simulink model "IEEE_34_node_2018a"  (R2018a)
settings: Solver=FixedStepDiscrete  StartTime=0.0  StopTime=0.01  RelTol=1e-3
InitFcn:
  | power_34NodeTestFeeder_init;
  | power_34NodeTestFeeder_loads_init;
  | %=============================
  | Vnom_ph_ph = 24900;
  | Vnom = 24900/sqrt(3);
  | Vnom1_ph_ph = 4160;
  | Vnom1 = 4160/sqrt(3);
  | Degrees_ph_ph_gen1 = 0;
  | Frequency = 60;
  | Apparent_power_gen1 = 2500e3;
  | SW1 = 0;
values from neighbouring files (symbols this model uses):
  Pa_802_806 = [1e-6 30 25]*1e3    [power_34NodeTestFeeder_loads_init.m]
  Pa_808_810 = 16e3    (= 16000)    [power_34NodeTestFeeder_loads_init.m]
  Pa_816_824 = [1e-6 5 1e-6]*1e3    [power_34NodeTestFeeder_loads_init.m]
  Pa_818_820 = 34e3    (= 34000)    [power_34NodeTestFeeder_loads_init.m]
  Pa_820_822 = 135e3    (= 135000)    [power_34NodeTestFeeder_loads_init.m]
  Pa_824_826 = 40e3    (= 40000)    [power_34NodeTestFeeder_loads_init.m]
  Pa_824_828 = [1e-6 1e-6 4]*1e3    [power_34NodeTestFeeder_loads_init.m]
  Pa_828_830 = [7 1e-6 1e-6]*1e3    [power_34NodeTestFeeder_loads_init.m]
  Pa_832_858 = [7 2 6]*1e3    [power_34NodeTestFeeder_loads_init.m]
  Pa_834_860 = [16 20 110]*1e3    [power_34NodeTestFeeder_loads_init.m]
  Pa_836_840 = [18 22 1e-6]*1e3    [power_34NodeTestFeeder_loads_init.m]
  Pa_842_844 = [9 1e-6 1e-6]*1e3    [power_34NodeTestFeeder_loads_init.m]
  Pa_844_846 = [1e-6 25 20]*1e3    [power_34NodeTestFeeder_loads_init.m]
  Pa_846_848 = [1e-6 23 1e-6]*1e3    [power_34NodeTestFeeder_loads_init.m]
  Pa_854_856 = 4e3    (= 4000)    [power_34NodeTestFeeder_loads_init.m]
  Pa_858_834 = [4 15 13]*1e3    [power_34NodeTestFeeder_loads_init.m]
  Pa_858_864 = 2e3    (= 2000)    [power_34NodeTestFeeder_loads_init.m]
  Pa_860_836 = [30 10 42]*1e3    [power_34NodeTestFeeder_loads_init.m]
  Pa_862_838 = 28e3    (= 28000)    [power_34NodeTestFeeder_loads_init.m]
  Pp_802_806 = [1e-6 15 14]*1e3    [power_34NodeTestFeeder_loads_init.m]
  Pp_808_810 = 8e3    (= 8000)    [power_34NodeTestFeeder_loads_init.m]
  Pp_816_824 = [1e-6 2 1e-6]*1e3    [power_34NodeTestFeeder_loads_init.m]
  Pp_818_820 = 17e3    (= 17000)    [power_34NodeTestFeeder_loads_init.m]
  Pp_820_822 = 70e3    (= 70000)    [power_34NodeTestFeeder_loads_init.m]
  Pp_824_826 = 20e3    (= 20000)    [power_34NodeTestFeeder_loads_init.m]
  Pp_824_828 = [1e-6 1e-6 2]*1e3    [power_34NodeTestFeeder_loads_init.m]
  Pp_828_830 = [3 1e-6 1e-6]*1e3    [power_34NodeTestFeeder_loads_init.m]
  Pp_832_858 = [3 1 3]*1e3    [power_34NodeTestFeeder_loads_init.m]
  Pp_834_860 = [8 10 55]*1e3    [power_34NodeTestFeeder_loads_init.m]
  Pp_836_840 = [9 11 1e-6]*1e3    [power_34NodeTestFeeder_loads_init.m]
  Pp_842_844 = [5 1e-6 1e-6]*1e3    [power_34NodeTestFeeder_loads_init.m]
  Pp_844_846 = [1e-6 12 11]*1e3    [power_34NodeTestFeeder_loads_init.m]
  Pp_846_848 = [1e-6 11 1e-6]*1e3    [power_34NodeTestFeeder_loads_init.m]
  Pp_854_856 = 2e3    (= 2000)    [power_34NodeTestFeeder_loads_init.m]
  Pp_858_834 = [2 8 7]*1e3    [power_34NodeTestFeeder_loads_init.m]
  Pp_858_864 = 1e3    (= 1000)    [power_34NodeTestFeeder_loads_init.m]
  Pp_860_836 = [15 6 22]*1e3    [power_34NodeTestFeeder_loads_init.m]
  Pp_862_838 = 14e3    (= 14000)    [power_34NodeTestFeeder_loads_init.m]
  V_802_806 = [1.047 1.048 1.048]    [power_34NodeTestFeeder_loads_init.m]
  V_808_810 = 1.014    [power_34NodeTestFeeder_loads_init.m]
  V_816_824 = [1.017 1.025 1.02]*sqrt(3)    [power_34NodeTestFeeder_loads_init.m]
  V_818_820 = 1.016    [power_34NodeTestFeeder_loads_init.m]
  V_820_822 = 0.993    [power_34NodeTestFeeder_loads_init.m]
  V_824_826 = 1.008    [power_34NodeTestFeeder_loads_init.m]
  V_824_828 = [1.008 1.016 1.012]    [power_34NodeTestFeeder_loads_init.m]
  V_828_830 = [1.007 1.015 1.011]    [power_34NodeTestFeeder_loads_init.m]
  V_830 = [0.989 0.998 0.994]*sqrt(3)    [power_34NodeTestFeeder_loads_init.m]
  V_832_858 = [1.036 1.035 1.036]*sqrt(3)    [power_34NodeTestFeeder_loads_init.m]
  V_834_860 = [1.031 1.029 1.031]*sqrt(3)    [power_34NodeTestFeeder_loads_init.m]
  V_836_840 = [1.03 1.029 1.031]*sqrt(3)    [power_34NodeTestFeeder_loads_init.m]
  V_840 = [1.03 1.029 1.031]    [power_34NodeTestFeeder_loads_init.m]
  V_842_844 = [1.031 1.029 1.031]    [power_34NodeTestFeeder_loads_init.m]
  V_844 = [1.031 1.029 1.031]    [power_34NodeTestFeeder_loads_init.m]
  V_844_846 = [1.031 1.029 1.031]    [power_34NodeTestFeeder_loads_init.m]
  V_846_848 = [1.031 1.029 1.031]    [power_34NodeTestFeeder_loads_init.m]
  V_848 = [1.031 1.029 1.031]*sqrt(3)    [power_34NodeTestFeeder_loads_init.m]
  V_854_856 = 0.998    [power_34NodeTestFeeder_loads_init.m]
  V_858_834 = [1.034 1.032 1.034]*sqrt(3)    [power_34NodeTestFeeder_loads_init.m]
  V_860 = [1.03 1.029 1.031]    [power_34NodeTestFeeder_loads_init.m]
  V_860_836 = [1.03 1.029 1.031]*sqrt(3)    [power_34NodeTestFeeder_loads_init.m]
  V_862_838 = 1.029    [power_34NodeTestFeeder_loads_init.m]
  V_890 = [0.917 0.924 0.918]*sqrt(3)    [power_34NodeTestFeeder_loads_init.m]
undefined symbols (not defined in the file or in its folder): Angle, C_300, C_301, C_302, C_303, C_304, Degrees_ph, ft2km, L_300, L_301, L_302, L_303, L_304, Magnitude, ph, ph_gen1, R_300, R_301, R_302, R_303, R_304, Vnom_ph
libraries: powerlib x148
(part 1 of 2)
settings Model: Creator=liyifu  LastModifiedBy=liyifu

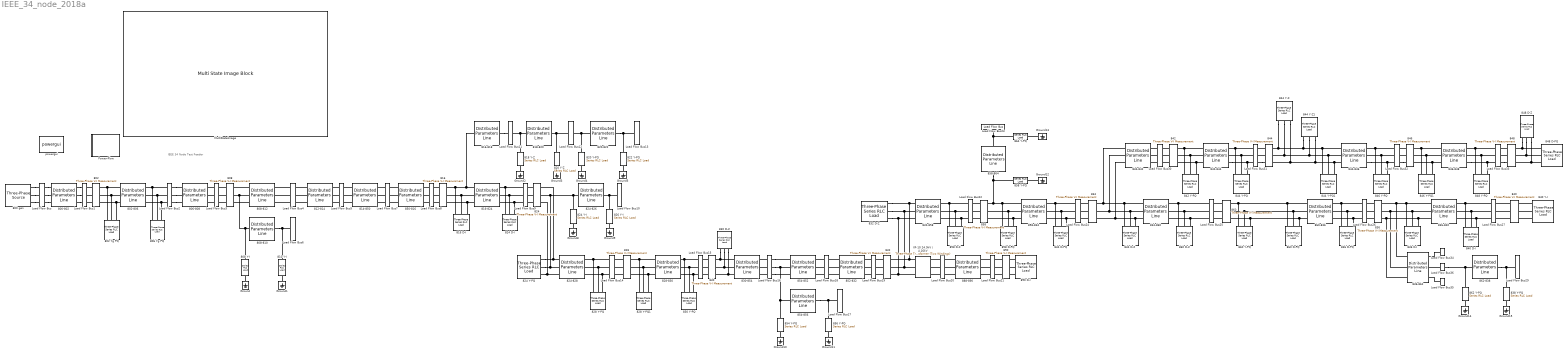
== system IEEE_34_node_2018a ==
  note: IEEE 34 Node Test Feeder
  800 gen : powerlib/Electrical Sources/Three-Phase Source  InternalConnection=Yg  VoltagePhases=on  Voltage=Vnom_ph-ph  PhaseAngle=Degrees_ph-ph_gen1  Voltage_phases=[1.05 1.05 1.05]*Vnom  PhaseAngles_phases=[0 -120 +120]  Frequency=Frequency  NonIdealSource=off  SpecifyImpedance=on  Resistance=0.8929  Inductance=16.58e-3  ShortCircuitLevel=Apparent_power_gen1  BaseVoltage=Vnom_ph_ph  XRratio=8  BusType=swing  Pref=10e3  Qref=0  Prefabc=[10e3, 10e3, 10e3]  Qrefabc=[0, 0, 0]  Qmin=-inf  Qmax=inf
      settings: SourceProductName=Simscape Electrical
  800-802 : powerlib/Elements/Distributed Parameters Line  Phases=3  Frequency=Frequency  Resistance=R_300  Inductance=L_300  Capacitance=C_300  Length=2580*ft2km  x1=[1249.92108084395 26131.4308609001 26009.0181767455;376.991118430775 376.991118430775 376.991118430775;1.94160573810255 0.298080075052811 1.87234868535801]  x2=[1257.44704241073 26098.7880044918 25982.8376072677;376.991118430775 376.991118430775 376.991118430775;1.94920053951311 0.296647201059818 1.87063909565862]  x3=[10.5571233758072 19.865376821896 26.3726391227777;376.991118430775 376.991118430775 376.991118430775;1.91729957078855 -0.988038774966991 0.129228047152116]  x4=[7.52563932812075 151.861194975018 136.408562693795;376.991118430775 376.991118430775 376.991118430775;-1.23536011490698 0.422640409864513 2.06263890147419]  x5=3.46223763231864e-06  V1=ones(3,3)  V2=ones(3,3)  I1=ones(3,3)  I2=ones(3,3)  nHarmo=1  Measurements=None
      settings: SourceProductName=Simscape Electrical
  802 : powerlib/Measurements/Three-Phase V-I Measurement  VoltageMeasurement=phase-to-ground  SetLabelV=on  LabelV=Vabc_802  Vpu=on  VpuLL=off  CurrentMeasurement=yes  SetLabelI=on  LabelI=Iabc_802  Ipu=on  Pbase=100e6  Vbase=Vnom_ph_ph  OutputType=Magnitude-Angle  PhasorSimulation=on  PSBequivalent=0
      settings: SourceProductName=Simscape Electrical
  802 Yg PQ : powerlib/Elements/Three-Phase Series RLC Load  LConnTagsString=A|B|C  Configuration=Y (grounded)  NominalVoltage=[  Vabc=V_802_806*Vnom  Vabcp=[1e3 1e3 1e3]  NominalFrequency=Frequency  UnbalancedPower=on  ActivePower=10e3  InductivePower=100  CapacitivePower=100  Pabc=Pa_802_806/2  QLabc=Pp_802_806/2  QCabc=Pn_802_806  Pabcp=[10e3 9e3 11e3]  QLabcp=[100 90 110]  QCabcp=[100 90 110]  Measurements=None  LoadType=constant PQ
      settings: SourceProductName=Simscape Electrical
      settings: AttributesFormatString=|
      | P= %<Pabc> W
      | Ql=%<QLabc> var
      | Qc=%<QCabc> var
  802-806 : powerlib/Elements/Distributed Parameters Line  Phases=3  Frequency=Frequency  Resistance=R_300  Inductance=L_300  Capacitance=C_300  Length=1730*ft2km  x1=[1257.44704241073 26098.7880044918 25982.8376072677;376.991118430775 376.991118430775 376.991118430775;1.94963055808353 0.297013701686642 1.87099846006617]  x2=[1262.34621488929 26077.2099428151 25966.1115766273;376.991118430775 376.991118430775 376.991118430775;1.95525458709618 0.296060428925334 1.86984860306052]  x3=[11.0972363781312 20.0856417950884 27.4183036232156;376.991118430775 376.991118430775 376.991118430775;1.97949951887063 -0.951655780421584 0.180146149087553]  x4=[8.04996886425621 150.996054293902 135.38429636786;376.991118430775 376.991118430775 376.991118430775;-1.15168297919955 0.422644259105267 2.07252538398702]  x5=2.32157794725242e-06  V1=ones(3,3)  V2=ones(3,3)  I1=ones(3,3)  I2=ones(3,3)  nHarmo=1  Measurements=None
      settings: SourceProductName=Simscape Electrical
  806 Yg PQ : powerlib/Elements/Three-Phase Series RLC Load  LConnTagsString=A|B|C  Configuration=Y (grounded)  NominalVoltage=[  Vabc=V_802_806*Vnom  Vabcp=[1e3 1e3 1e3]  NominalFrequency=Frequency  UnbalancedPower=on  ActivePower=10e3  InductivePower=100  CapacitivePower=100  Pabc=Pa_802_806/2  QLabc=Pp_802_806/2  QCabc=Pn_802_806  Pabcp=[10e3 9e3 11e3]  QLabcp=[100 90 110]  QCabcp=[100 90 110]  Measurements=None  LoadType=constant PQ
      settings: SourceProductName=Simscape Electrical
      settings: AttributesFormatString=|
      | P= %<Pabc> W
      | Ql=%<QLabc> var
      | Qc=%<QCabc> var
  806-808 : powerlib/Elements/Distributed Parameters Line  Phases=3  Frequency=Frequency  Resistance=R_300  Inductance=L_300  Capacitance=C_300  Length=32230*ft2km  x1=[1262.34621488929 26077.2099428151 25966.1115766273;376.991118430775 376.991118430775 376.991118430775;1.93982450898104 0.282909524080493 1.85695376255409]  x2=[1358.17424202311 25682.4173319928 25673.277529669;376.991118430775 376.991118430775 376.991118430775;2.04720135038634 0.265173822183593 1.83534880151853]  x3=[11.6001783263164 20.0026065935591 28.3021789406477;376.991118430775 376.991118430775 376.991118430775;2.01960794152478 -0.945866754158775 0.205483420334985]  x4=[8.46310811689409 146.878902947194 131.899465066813;376.991118430775 376.991118430775 376.991118430775;-1.11000249001825 0.39503335298076 2.05518911486961]  x5=4.32511313525697e-05  V1=ones(3,3)  V2=ones(3,3)  I1=ones(3,3)  I2=ones(3,3)  nHarmo=1  Measurements=None
      settings: SourceProductName=Simscape Electrical
  808 : powerlib/Measurements/Three-Phase V-I Measurement  VoltageMeasurement=phase-to-ground  SetLabelV=on  LabelV=Vabc_808  Vpu=on  VpuLL=off  CurrentMeasurement=yes  SetLabelI=on  LabelI=Iabc_808  Ipu=on  Pbase=100e6  Vbase=Vnom_ph_ph  OutputType=Magnitude-Angle  PhasorSimulation=on  PSBequivalent=0
      settings: SourceProductName=Simscape Electrical
  808 Y-I : powerlib/Elements/Series RLC Load  LConnTagsString=a  RConnTagsString=__new0  NominalVoltage=V_808_810*Vnom  NominalFrequency=Frequency  ActivePower=Pa_808_810/2  InductivePower=Pp_808_810/2  CapacitivePower=Pn_808_810  Setx0=off  InitialVoltage=0  SetiL0=off  InitialCurrent=0  Measurements=None  LoadType=constant I
      settings: SourceProductName=Simscape Electrical
      settings: AttributesFormatString=|
      | P=%<ActivePower> W
      | Ql=%<InductivePower> var
      | Qc=%<CapacitivePower> var
  808-810 : powerlib/Elements/Distributed Parameters Line  Phases=1  Frequency=Frequency  Resistance=R_303(2,2)  Inductance=L_303(2,2)  Capacitance=C_303(2,2)  Length=5804*ft2km  x1=[21119.0815149636;376.991118430775;-2.1231079032275]  x2=[21116.0661432003;376.991118430775;-2.12311859697996]  x3=[34.6870330793776;376.991118430775;-2.11449830893931]  x4=[36.2686607942877;376.991118430775;-2.13404984672294]  x5=7.30496713110932e-06  V1=ones(3,3)  V2=ones(3,3)  I1=ones(3,3)  I2=ones(3,3)  nHarmo=1  Measurements=None
      settings: SourceProductName=Simscape Electrical
  808-812 : powerlib/Elements/Distributed Parameters Line  Phases=3  Frequency=Frequency  Resistance=R_300  Inductance=L_300  Capacitance=C_300  Length=37500*ft2km  x1=[1358.17424202311 25682.4173319928 25673.277529669;376.991118430775 376.991118430775 376.991118430775;2.04453523524972 0.262901518297287 1.83312074219168]  x2=[1469.56545391947 25232.9999723138 25350.7201651836;376.991118430775 376.991118430775 376.991118430775;2.15905513464309 0.24225556988224 1.80744839784332]  x3=[11.6235578223822 19.8498204300557 29.7533327745572;376.991118430775 376.991118430775 376.991118430775;2.12229117690329 -0.959358085491786 0.191726647376344]  x4=[8.24346537921425 143.894679724776 130.199757058103;376.991118430775 376.991118430775 376.991118430775;-1.0079152617316 0.373661075158349 2.04266559454497]  x5=5.03232213999802e-05  V1=ones(3,3)  V2=ones(3,3)  I1=ones(3,3)  I2=ones(3,3)  nHarmo=1  Measurements=None
      settings: SourceProductName=Simscape Electrical
  810 Y-I : powerlib/Elements/Series RLC Load  LConnTagsString=a  RConnTagsString=__new0  NominalVoltage=V_808_810*Vnom  NominalFrequency=Frequency  ActivePower=Pa_808_810/2  InductivePower=Pp_808_810/2  CapacitivePower=Pn_808_810  Setx0=off  InitialVoltage=0  SetiL0=off  InitialCurrent=0  Measurements=None  LoadType=constant I
      settings: SourceProductName=Simscape Electrical
      settings: AttributesFormatString=|
      | P=%<ActivePower> W
      | Ql=%<InductivePower> var
      | Qc=%<CapacitivePower> var
  812-814 : powerlib/Elements/Distributed Parameters Line  Phases=3  Frequency=Frequency  Resistance=R_300  Inductance=L_300  Capacitance=C_300  Length=29730*ft2km  x1=[1469.56545391947 25232.9999723138 25350.7201651836;376.991118430775 376.991118430775 376.991118430775;2.16298601028095 0.245605816788614 1.81073341131004]  x2=[1569.41081620534 24879.7705046649 25102.4809009213;376.991118430775 376.991118430775 376.991118430775;2.24164443153353 0.228987694736397 1.79014174213356]  x3=[11.7818155561854 19.8150927770508 30.4752032611227;376.991118430775 376.991118430775 376.991118430775;2.14520492880805 -1.02022224188866 0.172242125340616]  x4=[8.14305816675558 143.018094733693 129.445364550441;376.991118430775 376.991118430775 376.991118430775;-1.01915035198126 0.362828883761539 2.03152246960354]  x5=3.98962499259043e-05  V1=ones(3,3)  V2=ones(3,3)  I1=ones(3,3)  I2=ones(3,3)  nHarmo=1  Measurements=None
      settings: SourceProductName=Simscape Electrical
  814-850 : powerlib/Elements/Distributed Parameters Line  Phases=3  Frequency=Frequency  Resistance=R_301  Inductance=L_301  Capacitance=C_301  Length=10*ft2km  x1=[669.7608170542 24884.6832259243 25125.0360475112;376.991118430775 376.991118430775 376.991118430775;-1.48243753027906 0.240288742139385 1.79965964476983]  x2=[669.74621388492 24884.491056861 25124.8873333344;376.991118430775 376.991118430775 376.991118430775;-1.4825443216982 0.24028222133131 1.79965138972404]  x3=[10.6357229600782 19.7192063960101 31.0303415847662;376.991118430775 376.991118430775 376.991118430775;2.23998543843376 -1.14786490473853 0.149955273352505]  x4=[11.8856149405288 142.657095608783 128.222738418226;376.991118430775 376.991118430775 376.991118430775;-0.969190911620163 0.376634213985134 2.04330765556362]  x5=1.37899021776565e-08  V1=ones(3,3)  V2=ones(3,3)  I1=ones(3,3)  I2=ones(3,3)  nHarmo=1  Measurements=None
      settings: SourceProductName=Simscape Electrical
  816 : powerlib/Measurements/Three-Phase V-I Measurement  VoltageMeasurement=phase-to-ground  SetLabelV=on  LabelV=Vabc_816  Vpu=on  VpuLL=off  CurrentMeasurement=yes  SetLabelI=on  LabelI=Iabc_816  Ipu=on  Pbase=100e6  Vbase=Vnom_ph_ph  OutputType=Magnitude-Angle  PhasorSimulation=on  PSBequivalent=0
      settings: SourceProductName=Simscape Electrical
  816 D-I : powerlib/Elements/Three-Phase Series RLC Load  LConnTagsString=A|B|C  Configuration=Delta  NominalVoltage=[  Vabc=[1.017 1.025 1.02]*sqrt(3)*Vnom  Vabcp=V_816_824*Vnom  NominalFrequency=Frequency  UnbalancedPower=on  ActivePower=10e3  InductivePower=100  CapacitivePower=100  Pabc=[0 30 25]*1e3/2  QLabc=[0 15 14]*1e3/2  QCabc=[0 0 0]  Pabcp=Pa_816_824/2  QLabcp=Pp_816_824/2  QCabcp=Pn_816_824  Measurements=None  LoadType=constant I
      settings: SourceProductName=Simscape Electrical
      settings: AttributesFormatString=|
      | P= %<Pabc> W
      | Ql=%<QLabc> var
      | Qc=%<QCabc> var
  816-818 : powerlib/Elements/Distributed Parameters Line  Phases=1  Frequency=Frequency  Resistance=R_302(1,1)  Inductance=L_302(1,1)  Capacitance=C_302(1,1)  Length=1710*ft2km  x1=[19869.2600721967;376.991118430775;-0.0627258903807259]  x2=[19851.3152704797;376.991118430775;-0.0627813243909014]  x3=[18.96809714002;376.991118430775;0.328260928650489]  x4=[49.9052646744321;376.991118430775;-0.208674404307824]  x5=2.15222153587128e-06  V1=ones(3,3)  V2=ones(3,3)  I1=ones(3,3)  I2=ones(3,3)  nHarmo=1  Measurements=None
      settings: SourceProductName=Simscape Electrical
  816-824 : powerlib/Elements/Distributed Parameters Line  Phases=3  Frequency=Frequency  Resistance=R_301  Inductance=L_301  Capacitance=C_301  Length=10210*ft2km  x1=[669.297297756189 24878.5341192423 25120.2778264531;376.991118430775 376.991118430775 376.991118430775;-1.49115978603529 0.235758468595441 1.79514164312775]  x2=[637.018239704485 24728.8928242446 24972.8766667643;376.991118430775 376.991118430775 376.991118430775;-1.49783953400905 0.228509227955325 1.7872262979359]  x3=[4.36968691100065 31.1847930023462 28.0632330952332;376.991118430775 376.991118430775 376.991118430775;0.850925211405672 -0.890665928385549 0.228148937955837]  x4=[5.46114690728559 132.850174983932 123.836134516563;376.991118430775 376.991118430775 376.991118430775;-2.10407022380879 0.442934898532415 2.01765281292941]  x5=1.40794901233873e-05  V1=ones(3,3)  V2=ones(3,3)  I1=ones(3,3)  I2=ones(3,3)  nHarmo=1  Measurements=None
      settings: SourceProductName=Simscape Electrical
  818 Y-Z : powerlib/Elements/Series RLC Load  LConnTagsString=a  RConnTagsString=__new0  NominalVoltage=V_818_820*Vnom  NominalFrequency=Frequency  ActivePower=Pa_818_820/2  InductivePower=Pp_818_820/2  CapacitivePower=Pn_818_820  Setx0=off  InitialVoltage=0  SetiL0=off  InitialCurrent=0  Measurements=None  LoadType=constant Z
      settings: SourceProductName=Simscape Electrical
      settings: AttributesFormatString=|
      | P=%<ActivePower> W
      | Ql=%<InductivePower> var
      | Qc=%<CapacitivePower> var
  818-820 : powerlib/Elements/Distributed Parameters Line  Phases=1  Frequency=Frequency  Resistance=R_302(1,1)  Inductance=L_302(1,1)  Capacitance=C_302(1,1)  Length=48150*ft2km  x1=[19851.3152704797;376.991118430775;-0.0848163820973309]  x2=[19391.8214982267;376.991118430775;-0.0858348834112547]  x3=[19.4193208414352;376.991118430775;0.247315554807652]  x4=[46.2735884766118;376.991118430775;-0.238948763434402]  x5=6.06020274574283e-05  V1=ones(3,3)  V2=ones(3,3)  I1=ones(3,3)  I2=ones(3,3)  nHarmo=1  Measurements=None
      settings: SourceProductName=Simscape Electrical
  820 Y-PQ : powerlib/Elements/Series RLC Load  LConnTagsString=a  RConnTagsString=__new0  NominalVoltage=V_820_822*Vnom  NominalFrequency=Frequency  ActivePower=Pa_820_822/2  InductivePower=Pp_820_822/2  CapacitivePower=Pn_820_822  Setx0=off  InitialVoltage=0  SetiL0=off  InitialCurrent=0  Measurements=None  LoadType=constant PQ
      settings: SourceProductName=Simscape Electrical
      settings: AttributesFormatString=|
      | P=%<ActivePower> W
      | Ql=%<InductivePower> var
      | Qc=%<CapacitivePower> var
  820 Y-Z : powerlib/Elements/Series RLC Load  LConnTagsString=a  RConnTagsString=__new0  NominalVoltage=V_818_820*Vnom  NominalFrequency=Frequency  ActivePower=Pa_818_820/2  InductivePower=Pp_818_820/2  CapacitivePower=Pn_818_820  Setx0=off  InitialVoltage=0  SetiL0=off  InitialCurrent=0  Measurements=None  LoadType=constant Z
      settings: SourceProductName=Simscape Electrical
      settings: AttributesFormatString=|
      | P=%<ActivePower> W
      | Ql=%<InductivePower> var
      | Qc=%<CapacitivePower> var
  820-822 : powerlib/Elements/Distributed Parameters Line  Phases=1  Frequency=Frequency  Resistance=R_302(1,1)  Inductance=L_302(1,1)  Capacitance=C_302(1,1)  Length=13740*ft2km  x1=[19391.8214982267;376.991118430775;-0.0695078735990618]  x2=[19332.7468483932;376.991118430775;-0.0695769850406438]  x3=[26.2226131335753;376.991118430775;0.048560985296662]  x4=[38.8103545088805;376.991118430775;-0.154709382906807]  x5=1.72932888320886e-05  V1=ones(3,3)  V2=ones(3,3)  I1=ones(3,3)  I2=ones(3,3)  nHarmo=1  Measurements=None
      settings: SourceProductName=Simscape Electrical
  822 Y-PQ : powerlib/Elements/Series RLC Load  LConnTagsString=a  RConnTagsString=__new0  NominalVoltage=V_820_822*Vnom  NominalFrequency=Frequency  ActivePower=Pa_820_822/2  InductivePower=Pp_820_822/2  CapacitivePower=Pn_820_822  Setx0=off  InitialVoltage=0  SetiL0=off  InitialCurrent=0  Measurements=None  LoadType=constant PQ
      settings: SourceProductName=Simscape Electrical
      settings: AttributesFormatString=|
      | P=%<ActivePower> W
      | Ql=%<InductivePower> var
      | Qc=%<CapacitivePower> var
  824 : powerlib/Measurements/Three-Phase V-I Measurement  VoltageMeasurement=phase-to-ground  SetLabelV=on  LabelV=Vabc_824  Vpu=on  VpuLL=off  CurrentMeasurement=yes  SetLabelI=on  LabelI=Iabc_824  Ipu=on  Pbase=100e6  Vbase=Vnom_ph_ph  OutputType=Magnitude-Angle  PhasorSimulation=on  PSBequivalent=0
      settings: SourceProductName=Simscape Electrical
  824 D-I : powerlib/Elements/Three-Phase Series RLC Load  LConnTagsString=A|B|C  Configuration=Delta  NominalVoltage=[  Vabc=[1.017 1.025 1.02]*sqrt(3)*Vnom  Vabcp=V_816_824*Vnom  NominalFrequency=Frequency  UnbalancedPower=on  ActivePower=10e3  InductivePower=100  CapacitivePower=100  Pabc=[0 30 25]*1e3/2  QLabc=[0 15 14]*1e3/2  QCabc=[0 0 0]  Pabcp=Pa_816_824/2  QLabcp=Pp_816_824/2  QCabcp=Pn_816_824  Measurements=None  LoadType=constant I
      settings: SourceProductName=Simscape Electrical
      settings: AttributesFormatString=|
      | P= %<Pabc> W
      | Ql=%<QLabc> var
      | Qc=%<QCabc> var
  824 Y-I : powerlib/Elements/Series RLC Load  LConnTagsString=a  RConnTagsString=__new0  NominalVoltage=V_824_826*Vnom  NominalFrequency=Frequency  ActivePower=Pa_824_826/2  InductivePower=Pp_824_826/2  CapacitivePower=Pn_824_826  Setx0=off  InitialVoltage=0  SetiL0=off  InitialCurrent=0  Measurements=None  LoadType=constant I
      settings: SourceProductName=Simscape Electrical
      settings: AttributesFormatString=|
      | P=%<ActivePower> W
      | Ql=%<InductivePower> var
      | Qc=%<CapacitivePower> var
  824 Y-PQ : powerlib/Elements/Three-Phase Series RLC Load  LConnTagsString=A|B|C  Configuration=Y (grounded)  NominalVoltage=[  Vabc=V_824_828*Vnom  Vabcp=[1.008 1.016 1.012]*Vnom  NominalFrequency=Frequency  UnbalancedPower=on  ActivePower=10e3  InductivePower=100  CapacitivePower=100  Pabc=Pa_824_828/2  QLabc=Pp_824_828/2  QCabc=Pn_824_828  Pabcp=[0 0 4]*1e3/2  QLabcp=[0 0 2]*1e3/2  QCabcp=[0 0 0]  Measurements=None  LoadType=constant PQ
      settings: SourceProductName=Simscape Electrical
      settings: AttributesFormatString=|
      | P= %<Pabc> W
      | Ql=%<QLabc> var
      | Qc=%<QCabc> var
  824-826 : powerlib/Elements/Distributed Parameters Line  Phases=1  Frequency=Frequency  Resistance=R_303(2,2)  Inductance=L_303(2,2)  Capacitance=C_303(2,2)  Length=3030*ft2km  x1=[20638.2047774201;376.991118430775;-2.17740572018252]  x2=[20634.23117712;376.991118430775;-2.1774123534692]  x3=[32.7859887350078;376.991118430775;-2.14899511081035]  x4=[36.7043804950352;376.991118430775;-2.20415074648027]  x5=3.81358552847368e-06  V1=ones(3,3)  V2=ones(3,3)  I1=ones(3,3)  I2=ones(3,3)  nHarmo=1  Measurements=None
      settings: SourceProductName=Simscape Electrical
  824-828 : powerlib/Elements/Distributed Parameters Line  Phases=3  Frequency=Frequency  Resistance=R_301  Inductance=L_301  Capacitance=C_301  Length=840*ft2km  x1=[637.018239704485 24728.8928242446 24972.8766667643;376.991118430775 376.991118430775 376.991118430775;-1.49296837961468 0.2324791474979 1.79113396244307]  x2=[635.673675429622 24717.2262249166 24961.4172077253;376.991118430775 376.991118430775 376.991118430775;-1.49430047635018 0.23190162251329 1.79046003567284]  x3=[2.25223495446006 31.9396656829298 30.8215706689758;376.991118430775 376.991118430775 376.991118430775;1.30619849621643 -0.81398677567269 0.255650052760832]  x4=[3.59155607107433 130.840713390775 123.949302221309;376.991118430775 376.991118430775 376.991118430775;-1.70546632028145 0.444876316743132 2.04175653602867]  x5=1.15835178292315e-06  V1=ones(3,3)  V2=ones(3,3)  I1=ones(3,3)  I2=ones(3,3)  nHarmo=1  Measurements=None
      settings: SourceProductName=Simscape Electrical
  826 Y-I : powerlib/Elements/Series RLC Load  LConnTagsString=a  RConnTagsString=__new0  NominalVoltage=V_824_826*Vnom  NominalFrequency=Frequency  ActivePower=Pa_824_826/2  InductivePower=Pp_824_826/2  CapacitivePower=Pn_824_826  Setx0=off  InitialVoltage=0  SetiL0=off  InitialCurrent=0  Measurements=None  LoadType=constant I
      settings: SourceProductName=Simscape Electrical
      settings: AttributesFormatString=|
      | P=%<ActivePower> W
      | Ql=%<InductivePower> var
      | Qc=%<CapacitivePower> var
  828 : powerlib/Measurements/Three-Phase V-I Measurement  VoltageMeasurement=phase-to-ground  SetLabelV=on  LabelV=Vabc_828  Vpu=on  VpuLL=off  CurrentMeasurement=yes  SetLabelI=on  LabelI=Iabc_828  Ipu=on  Pbase=100e6  Vbase=Vnom_ph_ph  OutputType=Magnitude-Angle  PhasorSimulation=on  PSBequivalent=0
      settings: SourceProductName=Simscape Electrical
  828 Y-PQ : powerlib/Elements/Three-Phase Series RLC Load  LConnTagsString=A|B|C  Configuration=Y (grounded)  NominalVoltage=[  Vabc=V_824_828*Vnom  Vabcp=[1.008 1.016 1.012]*Vnom  NominalFrequency=Frequency  UnbalancedPower=on  ActivePower=10e3  InductivePower=100  CapacitivePower=100  Pabc=Pa_824_828/2  QLabc=Pp_824_828/2  QCabc=Pn_824_828  Pabcp=[0 0 4]*1e3/2  QLabcp=[0 0 2]*1e3/2  QCabcp=[0 0 0]  Measurements=None  LoadType=constant PQ
      settings: SourceProductName=Simscape Electrical
      settings: AttributesFormatString=|
      | P= %<Pabc> W
      | Ql=%<QLabc> var
      | Qc=%<QCabc> var
  828 Y-PQ1 : powerlib/Elements/Three-Phase Series RLC Load  LConnTagsString=A|B|C  Configuration=Y (grounded)  NominalVoltage=[  Vabc=V_828_830*Vnom  Vabcp=[1.008 1.016 1.012]*Vnom  NominalFrequency=Frequency  UnbalancedPower=on  ActivePower=10e3  InductivePower=100  CapacitivePower=100  Pabc=Pa_828_830/2  QLabc=Pp_828_830/2  QCabc=Pn_828_830  Pabcp=[0 0 4]*1e3/2  QLabcp=[0 0 2]*1e3/2  QCabcp=[0 0 0]  Measurements=None  LoadType=constant PQ
      settings: SourceProductName=Simscape Electrical
      settings: AttributesFormatString=|
      | P= %<Pabc> W
      | Ql=%<QLabc> var
      | Qc=%<QCabc> var
  828-830 : powerlib/Elements/Distributed Parameters Line  Phases=3  Frequency=Frequency  Resistance=R_301  Inductance=L_301  Capacitance=C_301  Length=20440*ft2km  x1=[635.673675429622 24717.2262249166 24961.4172077253;376.991118430775 376.991118430775 376.991118430775;-1.50448987081439 0.223597415145683 1.78228605228538]  x2=[601.287036352134 24436.8994336664 24686.5156314332;376.991118430775 376.991118430775 376.991118430775;-1.53587251532522 0.209428113553337 1.76580414802682]  x3=[2.31969871934651 31.7720570459509 30.5873085234824;376.991118430775 376.991118430775 376.991118430775;1.21736133349944 -0.830325240506862 0.24642590112485]  x4=[3.59292222973066 128.054918862299 121.560613327383;376.991118430775 376.991118430775 376.991118430775;-1.77870237402968 0.428167673220865 2.02387530834998]  x5=2.81865600511299e-05  V1=ones(3,3)  V2=ones(3,3)  I1=ones(3,3)  I2=ones(3,3)  nHarmo=1  Measurements=None
      settings: SourceProductName=Simscape Electrical
  830 : powerlib/Measurements/Three-Phase V-I Measurement  VoltageMeasurement=phase-to-ground  SetLabelV=on  LabelV=Vabc_830  Vpu=on  VpuLL=off  CurrentMeasurement=yes  SetLabelI=on  LabelI=Iabc_830  Ipu=on  Pbase=100e6  Vbase=Vnom_ph_ph  OutputType=Magnitude-Angle  PhasorSimulation=on  PSBequivalent=0
      settings: SourceProductName=Simscape Electrical
  830 D-Z : powerlib/Elements/Three-Phase Series RLC Load  LConnTagsString=A|B|C  Configuration=Delta  NominalVoltage=[  Vabc=[1.017 1.025 1.02]*sqrt(3)*Vnom  Vabcp=V_830*Vnom  NominalFrequency=Frequency  UnbalancedPower=on  ActivePower=10e3  InductivePower=100  CapacitivePower=100  Pabc=[0 30 25]*1e3/2  QLabc=[0 15 14]*1e3/2  QCabc=[0 0 0]  Pabcp=Pa_830  QLabcp=Pp_830  QCabcp=Pn_830  Measurements=None  LoadType=constant Z
      settings: SourceProductName=Simscape Electrical
      settings: AttributesFormatString=|
      | P= %<Pabc> W
      | Ql=%<QLabc> var
      | Qc=%<QCabc> var
  830 Y-PQ : powerlib/Elements/Three-Phase Series RLC Load  LConnTagsString=A|B|C  Configuration=Y (grounded)  NominalVoltage=[  Vabc=V_828_830*Vnom  Vabcp=[1.008 1.016 1.012]*Vnom  NominalFrequency=Frequency  UnbalancedPower=on  ActivePower=10e3  InductivePower=100  CapacitivePower=100  Pabc=Pa_828_830/2  QLabc=Pp_828_830/2  QCabc=Pn_828_830  Pabcp=[0 0 4]*1e3/2  QLabcp=[0 0 2]*1e3/2  QCabcp=[0 0 0]  Measurements=None  LoadType=constant PQ
      settings: SourceProductName=Simscape Electrical
      settings: AttributesFormatString=|
      | P= %<Pabc> W
      | Ql=%<QLabc> var
      | Qc=%<QCabc> var
  830-854 : powerlib/Elements/Distributed Parameters Line  Phases=3  Frequency=Frequency  Resistance=R_301  Inductance=L_301  Capacitance=C_301  Length=520*ft2km  x1=[601.287036352134 24436.8994336664 24686.5156314332;376.991118430775 376.991118430775 376.991118430775;-1.52551676340037 0.217867899816742 1.77411158420428]  x2=[600.415344439585 24430.2182967214 24679.9493391831;376.991118430775 376.991118430775 376.991118430775;-1.52617739951622 0.217500171996073 1.77369575342487]  x3=[2.24837479458079 34.3986849322115 31.5997630877242;376.991118430775 376.991118430775 376.991118430775;1.10573653139527 -0.8187450702249 0.306471269019442]  x4=[3.4533394454739 128.179899166488 120.709427985989;376.991118430775 376.991118430775 376.991118430775;-1.84935582786226 0.450612810902678 2.03721471359926]  x5=7.17074913238139e-07  V1=ones(3,3)  V2=ones(3,3)  I1=ones(3,3)  I2=ones(3,3)  nHarmo=1  Measurements=None
      settings: SourceProductName=Simscape Electrical
  832 : powerlib/Measurements/Three-Phase V-I Measurement  VoltageMeasurement=phase-to-ground  SetLabelV=on  LabelV=Vabc_832  Vpu=on  VpuLL=off  CurrentMeasurement=yes  SetLabelI=on  LabelI=Iabc_832  Ipu=on  Pbase=100e6  Vbase=Vnom_ph_ph  OutputType=Magnitude-Angle  PhasorSimulation=on  PSBequivalent=0
      settings: SourceProductName=Simscape Electrical
  832 D-Z : powerlib/Elements/Three-Phase Series RLC Load  LConnTagsString=A|B|C  Configuration=Delta  NominalVoltage=[  Vabc=[1.017 1.025 1.02]*sqrt(3)*Vnom  Vabcp=V_832_858*Vnom  NominalFrequency=Frequency  UnbalancedPower=on  ActivePower=10e3  InductivePower=100  CapacitivePower=100  Pabc=[0 30 25]*1e3/2  QLabc=[0 15 14]*1e3/2  QCabc=[0 0 0]  Pabcp=Pa_832_858/2  QLabcp=Pp_832_858/2  QCabcp=Pn_832_858  Measurements=None  LoadType=constant Z
      settings: SourceProductName=Simscape Electrical
      settings: AttributesFormatString=|
      | P= %<Pabc> W
      | Ql=%<QLabc> var
      | Qc=%<QCabc> var
  832-858 : powerlib/Elements/Distributed Parameters Line  Phases=3  Frequency=Frequency  Resistance=R_301  Inductance=L_301  Capacitance=C_301  Length=4900*ft2km  x1=[544.297090319122 23962.1950623007 24225.8849285826;376.991118430775 376.991118430775 376.991118430775;-1.57363040145649 0.189493419417186 1.74208300295025]  x2=[538.916079582122 23936.381353331 24203.4007325891;376.991118430775 376.991118430775 376.991118430775;-1.57527517916447 0.185868800435926 1.73805296350572]  x3=[1.29723917616971 52.8684457924366 47.3954754221382;376.991118430775 376.991118430775 376.991118430775;0.622930723400035 -0.656927709691266 0.637340252599691]  x4=[2.20825884422358 111.101810545025 104.723116464672;376.991118430775 376.991118430775 376.991118430775;-2.07115911053738 0.550064652386419 2.15459413769142]  x5=6.7570520670517e-06  V1=ones(3,3)  V2=ones(3,3)  I1=ones(3,3)  I2=ones(3,3)  nHarmo=1  Measurements=None
      settings: SourceProductName=Simscape Electrical
  834 : powerlib/Measurements/Three-Phase V-I Measurement  VoltageMeasurement=phase-to-ground  SetLabelV=on  LabelV=Vabc_834  Vpu=on  VpuLL=off  CurrentMeasurement=yes  SetLabelI=on  LabelI=Iabc_834  Ipu=on  Pbase=100e6  Vbase=Vnom_ph_ph  OutputType=Magnitude-Angle  PhasorSimulation=on  PSBequivalent=0
      settings: SourceProductName=Simscape Electrical
  834 D-PQ : powerlib/Elements/Three-Phase Series RLC Load  LConnTagsString=A|B|C  Configuration=Delta  NominalVoltage=[  Vabc=[1.017 1.025 1.02]*sqrt(3)*Vnom  Vabcp=V_858_834*Vnom  NominalFrequency=Frequency  UnbalancedPower=on  ActivePower=10e3  InductivePower=100  CapacitivePower=100  Pabc=[0 30 25]*1e3/2  QLabc=[0 15 14]*1e3/2  QCabc=[0 0 0]  Pabcp=Pa_858_834/2  QLabcp=Pp_858_834/2  QCabcp=Pn_858_834  Measurements=None  LoadType=constant PQ
      settings: SourceProductName=Simscape Electrical
      settings: AttributesFormatString=|
      | P= %<Pabc> W
      | Ql=%<QLabc> var
      | Qc=%<QCabc> var
  834 D-Z : powerlib/Elements/Three-Phase Series RLC Load  LConnTagsString=A|B|C  Configuration=Delta  NominalVoltage=[  Vabc=[1.017 1.025 1.02]*sqrt(3)*Vnom  Vabcp=V_834_860*Vnom  NominalFrequency=Frequency  UnbalancedPower=on  ActivePower=10e3  InductivePower=100  CapacitivePower=100  Pabc=[0 30 25]*1e3/2  QLabc=[0 15 14]*1e3/2  QCabc=[0 0 0]  Pabcp=Pa_834_860/2  QLabcp=Pp_834_860/2  QCabcp=Pn_834_860  Measurements=None  LoadType=constant Z
      settings: SourceProductName=Simscape Electrical
      settings: AttributesFormatString=|
      | P= %<Pabc> W
      | Ql=%<QLabc> var
      | Qc=%<QCabc> var
  834-842 : powerlib/Elements/Distributed Parameters Line  Phases=3  Frequency=Frequency  Resistance=R_301  Inductance=L_301  Capacitance=C_301  Length=280*ft2km  x1=[532.488097890621 23907.9048332495 24179.347575776;376.991118430775 376.991118430775 376.991118430775;-1.5738010972037 0.183503521668224 1.73519817574279]  x2=[532.560098856686 23908.1567468527 24179.8968067617;376.991118430775 376.991118430775 376.991118430775;-1.57375382845556 0.183279337224048 1.73497886153928]  x3=[0.972485409830439 70.724344430212 62.0978591081052;376.991118430775 376.991118430775 376.991118430775;-1.77765362434399 -0.614329731124174 0.834703061723499]  x4=[0.288188518469659 103.091898225527 92.6081132341689;376.991118430775 376.991118430775 376.991118430775;-0.822017371184678 0.696581277115551 2.28820569141929]  x5=3.86117260974383e-07  V1=ones(3,3)  V2=ones(3,3)  I1=ones(3,3)  I2=ones(3,3)  nHarmo=1  Measurements=None
      settings: SourceProductName=Simscape Electrical
  834-860 : powerlib/Elements/Distributed Parameters Line  Phases=3  Frequency=Frequency  Resistance=R_301  Inductance=L_301  Capacitance=C_301  Length=2020*ft2km  x1=[532.488097890621 23907.9048332495 24179.347575776;376.991118430775 376.991118430775 376.991118430775;-1.57470566589593 0.182766311422324 1.73447252619717]  x2=[529.898068973042 23898.4588495649 24170.0388321035;376.991118430775 376.991118430775 376.991118430775;-1.57474565502375 0.182826368932349 1.73445969410462]  x3=[1.63328036165873 58.7099677379436 47.5606280616576;376.991118430775 376.991118430775 376.991118430775;0.488910014175005 0.307610071221618 1.85359151611361]  x4=[2.40930708204933 81.0863982856748 70.2473653685472;376.991118430775 376.991118430775 376.991118430775;-2.21508285043218 0.0918009452492619 1.65321083575864]  x5=2.78556023988662e-06  V1=ones(3,3)  V2=ones(3,3)  I1=ones(3,3)  I2=ones(3,3)  nHarmo=1  Measurements=None
      settings: SourceProductName=Simscape Electrical
  836 : powerlib/Measurements/Three-Phase V-I Measurement  VoltageMeasurement=phase-to-ground  SetLabelV=on  LabelV=Vabc_836  Vpu=on  VpuLL=off  CurrentMeasurement=yes  SetLabelI=on  LabelI=Iabc_836  Ipu=on  Pbase=100e6  Vbase=Vnom_ph_ph  OutputType=Magnitude-Angle  PhasorSimulation=on  PSBequivalent=0
      settings: SourceProductName=Simscape Electrical
  836 D-I : powerlib/Elements/Three-Phase Series RLC Load  LConnTagsString=A|B|C  Configuration=Delta  NominalVoltage=[  Vabc=[1.017 1.025 1.02]*sqrt(3)*Vnom  Vabcp=V_836_840*Vnom  NominalFrequency=Frequency  UnbalancedPower=on  ActivePower=10e3  InductivePower=100  CapacitivePower=100  Pabc=[0 30 25]*1e3/2  QLabc=[0 15 14]*1e3/2  QCabc=[0 0 0]  Pabcp=Pa_836_840/2  QLabcp=Pp_836_840/2  QCabcp=Pn_836_840  Measurements=None  LoadType=constant I
      settings: SourceProductName=Simscape Electrical
      settings: AttributesFormatString=|
      | P= %<Pabc> W
      | Ql=%<QLabc> var
      | Qc=%<QCabc> var
  836 D-PQ : powerlib/Elements/Three-Phase Series RLC Load  LConnTagsString=A|B|C  Configuration=Delta  NominalVoltage=[  Vabc=[1.017 1.025 1.02]*sqrt(3)*Vnom  Vabcp=V_860_836*Vnom  NominalFrequency=Frequency  UnbalancedPower=on  ActivePower=10e3  InductivePower=100  CapacitivePower=100  Pabc=[0 30 25]*1e3/2  QLabc=[0 15 14]*1e3/2  QCabc=[0 0 0]  Pabcp=Pa_860_836/2  QLabcp=Pp_860_836/2  QCabcp=Pn_860_836  Measurements=None  LoadType=constant PQ
      settings: SourceProductName=Simscape Electrical
      settings: AttributesFormatString=|
      | P= %<Pabc> W
      | Ql=%<QLabc> var
      | Qc=%<QCabc> var
  836-840 : powerlib/Elements/Distributed Parameters Line  Phases=3  Frequency=Frequency  Resistance=R_301  Inductance=L_301  Capacitance=C_301  Length=860*ft2km  x1=[526.843358587077 23892.7809998017 24164.7359964069;376.991118430775 376.991118430775 376.991118430775;-1.57308914165041 0.183273286351239 1.73500447386127]  x2=[526.803514703196 23892.1759032398 24164.0726411531;376.991118430775 376.991118430775 376.991118430775;-1.57311376940977 0.183271808368671 1.73501207127654]  x3=[0.510845372924359 67.6621593415957 57.059033430526;376.991118430775 376.991118430775 376.991118430775;-1.5015887629287 0.193756770923144 1.76168035684478]  x4=[0.64168752557632 71.3999314397603 60.2490456702427;376.991118430775 376.991118430775 376.991118430775;-1.63041606492187 0.172982288304378 1.70939949530344]  x5=1.18593158727846e-06  V1=ones(3,3)  V2=ones(3,3)  I1=ones(3,3)  I2=ones(3,3)  nHarmo=1  Measurements=None
      settings: SourceProductName=Simscape Electrical
  836-862 : powerlib/Elements/Distributed Parameters Line  Phases=3  Frequency=Frequency  Resistance=R_301  Inductance=L_301  Capacitance=C_301  Length=280*ft2km  x1=[526.843358587077 23892.7809998017 24164.7359964069;376.991118430775 376.991118430775 376.991118430775;-1.572787618753 0.183519023099872 1.73524635704314]  x2=[526.548353531827 23892.6530875428 24164.6254067925;376.991118430775 376.991118430775 376.991118430775;-1.57263196771958 0.183514334830567 1.73525075784239]  x3=[1.5114465772424 67.9042329654386 58.2102323915336;376.991118430775 376.991118430775 376.991118430775;0.128516773467724 0.176124880592363 1.75998009197564]  x4=[2.01487486252301 71.211679623214 59.1340381995524;376.991118430775 376.991118430775 376.991118430775;-2.41146845447374 0.190449273339831 1.71078759688826]  x5=3.86117260974383e-07  V1=ones(3,3)  V2=ones(3,3)  I1=ones(3,3)  I2=ones(3,3)  nHarmo=1  Measurements=None
      settings: SourceProductName=Simscape Electrical
  838 Y-PQ : powerlib/Elements/Series RLC Load  LConnTagsString=a  RConnTagsString=__new0  NominalVoltage=V_862_838*Vnom  NominalFrequency=Frequency  ActivePower=Pa_862_838/2  InductivePower=Pp_862_838/2  CapacitivePower=Pn_862_838  Setx0=off  InitialVoltage=0  SetiL0=off  InitialCurrent=0  Measurements=None  LoadType=constant PQ
      settings: SourceProductName=Simscape Electrical
      settings: AttributesFormatString=|
      | P=%<ActivePower> W
      | Ql=%<InductivePower> var
      | Qc=%<CapacitivePower> var
  840 : powerlib/Measurements/Three-Phase V-I Measurement  VoltageMeasurement=phase-to-ground  SetLabelV=on  LabelV=Vabc_840  Vpu=on  VpuLL=off  CurrentMeasurement=yes  SetLabelI=on  LabelI=Iabc_840  Ipu=on  Pbase=100e6  Vbase=Vnom_ph_ph  OutputType=Magnitude-Angle  PhasorSimulation=on  PSBequivalent=0
      settings: SourceProductName=Simscape Electrical
  840 D-I : powerlib/Elements/Three-Phase Series RLC Load  LConnTagsString=A|B|C  Configuration=Delta  NominalVoltage=[  Vabc=[1.017 1.025 1.02]*sqrt(3)*Vnom  Vabcp=V_836_840*Vnom  NominalFrequency=Frequency  UnbalancedPower=on  ActivePower=10e3  InductivePower=100  CapacitivePower=100  Pabc=[0 30 25]*1e3/2  QLabc=[0 15 14]*1e3/2  QCabc=[0 0 0]  Pabcp=Pa_836_840/2  QLabcp=Pp_836_840/2  QCabcp=Pn_836_840  Measurements=None  LoadType=constant I
      settings: SourceProductName=Simscape Electrical
      settings: AttributesFormatString=|
      | P= %<Pabc> W
      | Ql=%<QLabc> var
      | Qc=%<QCabc> var
  840 Y-I : powerlib/Elements/Three-Phase Series RLC Load  LConnTagsString=A|B|C  Configuration=Y (grounded)  NominalVoltage=1000  Vabc=V_840*Vnom  Vabcp=[1e3 1e3 1e3]  NominalFrequency=Frequency  UnbalancedPower=on  ActivePower=10e3  InductivePower=100  CapacitivePower=100  Pabc=Pa_840  QLabc=Pp_840  QCabc=Pn_840  Pabcp=[10e3 9e3 11e3]  QLabcp=[100 90 110]  QCabcp=[100 90 110]  Measurements=None  LoadType=constant I
      settings: SourceProductName=Simscape Electrical
      settings: AttributesFormatString=|
      | P= %<Pabc> W
      | Ql=%<QLabc> var
      | Qc=%<QCabc> var
  842 : powerlib/Measurements/Three-Phase V-I Measurement  VoltageMeasurement=phase-to-ground  SetLabelV=on  LabelV=Vabc_842  Vpu=on  VpuLL=off  CurrentMeasurement=yes  SetLabelI=on  LabelI=Iabc_842  Ipu=on  Pbase=100e6  Vbase=Vnom_ph_ph  OutputType=Magnitude-Angle  PhasorSimulation=on  PSBequivalent=0
      settings: SourceProductName=Simscape Electrical
  842 Y-PQ : powerlib/Elements/Three-Phase Series RLC Load  LConnTagsString=A|B|C  Configuration=Y (grounded)  NominalVoltage=[  Vabc=V_842_844*Vnom  Vabcp=[1.031 1.029 1.031]*sqrt(3)*Vnom  NominalFrequency=Frequency  UnbalancedPower=on  ActivePower=10e3  InductivePower=100  CapacitivePower=100  Pabc=Pa_842_844/2  QLabc=Pp_842_844/2  QCabc=Pn_842_844  Pabcp=[16 20 110]*1e3/2  QLabcp=[8 10 55]*1e3/2  QCabcp=[0 0 0]  Measurements=None  LoadType=constant PQ
      settings: SourceProductName=Simscape Electrical
      settings: AttributesFormatString=|
      | P= %<Pabc> W
      | Ql=%<QLabc> var
      | Qc=%<QCabc> var
  842-844 : powerlib/Elements/Distributed Parameters Line  Phases=3  Frequency=Frequency  Resistance=R_301  Inductance=L_301  Capacitance=C_301  Length=1350*ft2km  x1=[532.560098856686 23908.1567468527 24179.8968067617;376.991118430775 376.991118430775 376.991118430775;-1.57431008621457 0.182825995291225 1.73453262877272]  x2=[532.858804830353 23909.5344403469 24182.5702844361;376.991118430775 376.991118430775 376.991118430775;-1.57364231122933 0.18174309367146 1.73347760584717]  x3=[1.11121270955152 71.024975502821 62.0592829213778;376.991118430775 376.991118430775 376.991118430775;-1.55136832727018 -0.61506623607051 0.835624985905007]  x4=[0.0578291861142763 102.887673684504 92.4200514058512;376.991118430775 376.991118430775 376.991118430775;-2.03117715282753 0.698439307112783 2.28667687424365]  x5=1.86163679398363e-06  V1=ones(3,3)  V2=ones(3,3)  I1=ones(3,3)  I2=ones(3,3)  nHarmo=1  Measurements=None
      settings: SourceProductName=Simscape Electrical
  844 : powerlib/Measurements/Three-Phase V-I Measurement  VoltageMeasurement=phase-to-ground  SetLabelV=on  LabelV=Vabc_844  Vpu=on  VpuLL=off  CurrentMeasurement=yes  SetLabelI=on  LabelI=Iabc_844  Ipu=on  Pbase=100e6  Vbase=Vnom_ph_ph  OutputType=Magnitude-Angle  PhasorSimulation=on  PSBequivalent=0
      settings: SourceProductName=Simscape Electrical
  844 Y-PQ : powerlib/Elements/Three-Phase Series RLC Load  LConnTagsString=A|B|C  Configuration=Y (grounded)  NominalVoltage=[  Vabc=V_842_844*Vnom  Vabcp=[1.031 1.029 1.031]*sqrt(3)*Vnom  NominalFrequency=Frequency  UnbalancedPower=on  ActivePower=10e3  InductivePower=100  CapacitivePower=100  Pabc=Pa_842_844/2  QLabc=Pp_842_844/2  QCabc=Pn_842_844  Pabcp=[16 20 110]*1e3/2  QLabcp=[8 10 55]*1e3/2  QCabcp=[0 0 0]  Measurements=None  LoadType=constant PQ
      settings: SourceProductName=Simscape Electrical
      settings: AttributesFormatString=|
      | P= %<Pabc> W
      | Ql=%<QLabc> var
      | Qc=%<QCabc> var
  844 Y-PQ1 : powerlib/Elements/Three-Phase Series RLC Load  LConnTagsString=A|B|C  Configuration=Y (grounded)  NominalVoltage=[  Vabc=V_844_846*Vnom  Vabcp=[1.031 1.029 1.031]*sqrt(3)*Vnom  NominalFrequency=Frequency  UnbalancedPower=on  ActivePower=10e3  InductivePower=100  CapacitivePower=100  Pabc=Pa_844_846/2  QLabc=Pp_844_846/2  QCabc=Pn_844_846  Pabcp=[16 20 110]*1e3/2  QLabcp=[8 10 55]*1e3/2  QCabcp=[0 0 0]  Measurements=None  LoadType=constant PQ
      settings: SourceProductName=Simscape Electrical
      settings: AttributesFormatString=|
      | P= %<Pabc> W
      | Ql=%<QLabc> var
      | Qc=%<QCabc> var
  844 Y-Z : powerlib/Elements/Three-Phase Series RLC Load  LConnTagsString=A|B|C  Configuration=Y (grounded)  NominalVoltage=[  Vabc=V_844*Vnom  Vabcp=[1.031 1.029 1.031]*sqrt(3)*Vnom  NominalFrequency=Frequency  UnbalancedPower=on  ActivePower=10e3  InductivePower=100  CapacitivePower=100  Pabc=Pa_844  QLabc=Pp_844  QCabc=[0 0 0]  Pabcp=[16 20 110]*1e3/2  QLabcp=[8 10 55]*1e3/2  QCabcp=[0 0 0]  Measurements=Branch voltages and currents  LoadType=constant Z
      settings: SourceProductName=Simscape Electrical
      settings: AttributesFormatString=|
      | P= %<Pabc> W
      | Ql=%<QLabc> var
      | Qc=%<QCabc> var
  844 Y-Z1 : powerlib/Elements/Three-Phase Series RLC Load  LConnTagsString=A|B|C  Configuration=Y (grounded)  NominalVoltage=[  Vabc="[1  1  1]*Vnom"  Vabcp=[1.031 1.029 1.031]*sqrt(3)*Vnom  NominalFrequency=Frequency  UnbalancedPower=on  ActivePower=10e3  InductivePower=100  CapacitivePower=100  Pabc=[0 0 0]  QLabc=[0 0 0]  QCabc=Pn_844  Pabcp=[16 20 110]*1e3/2  QLabcp=[8 10 55]*1e3/2  QCabcp=[0 0 0]  Measurements=None  LoadType=constant Z
      settings: SourceProductName=Simscape Electrical
      settings: AttributesFormatString=|
      | P= %<Pabc> W
      | Ql=%<QLabc> var
      | Qc=%<QCabc> var
  844-846 : powerlib/Elements/Distributed Parameters Line  Phases=3  Frequency=Frequency  Resistance=R_301  Inductance=L_301  Capacitance=C_301  Length=3640*ft2km  x1=[532.858804830353 23909.5344403469 24182.5702844361;376.991118430775 376.991118430775 376.991118430775;-1.57483280680704 0.180772857198408 1.73252258431874]  x2=[535.070490121194 23931.5919189507 24208.9096649864;376.991118430775 376.991118430775 376.991118430775;-1.57278120499495 0.178203802242893 1.73006425383981]  x3=[1.60111301073845 82.661810298897 73.5768260539317;376.991118430775 376.991118430775 376.991118430775;-1.80909615202913 -0.481352973103418 0.999270332209357]  x4=[0.540815386363668 89.4049931081928 79.4747052136032;376.991118430775 376.991118430775 376.991118430775;0.808859247217282 0.781483169594141 2.39704928823832]  x5=5.01952439266698e-06  V1=ones(3,3)  V2=ones(3,3)  I1=ones(3,3)  I2=ones(3,3)  nHarmo=1  Measurements=None
      settings: SourceProductName=Simscape Electrical
  846 : powerlib/Measurements/Three-Phase V-I Measurement  VoltageMeasurement=phase-to-ground  SetLabelV=on  LabelV=Vabc_846  Vpu=on  VpuLL=off  CurrentMeasurement=yes  SetLabelI=on  LabelI=Iabc_846  Ipu=on  Pbase=100e6  Vbase=Vnom_ph_ph  OutputType=Magnitude-Angle  PhasorSimulation=on  PSBequivalent=0
      settings: SourceProductName=Simscape Electrical
  846 Y-PQ : powerlib/Elements/Three-Phase Series RLC Load  LConnTagsString=A|B|C  Configuration=Y (grounded)  NominalVoltage=[  Vabc=V_844_846*Vnom  Vabcp=[1.031 1.029 1.031]*sqrt(3)*Vnom  NominalFrequency=Frequency  UnbalancedPower=on  ActivePower=10e3  InductivePower=100  CapacitivePower=100  Pabc=Pa_844_846/2  QLabc=Pp_844_846/2  QCabc=Pn_844_846  Pabcp=[16 20 110]*1e3/2  QLabcp=[8 10 55]*1e3/2  QCabcp=[0 0 0]  Measurements=None  LoadType=constant PQ
      settings: SourceProductName=Simscape Electrical
      settings: AttributesFormatString=|
      | P= %<Pabc> W
      | Ql=%<QLabc> var
      | Qc=%<QCabc> var
  846 Y-PQ1 : powerlib/Elements/Three-Phase Series RLC Load  LConnTagsString=A|B|C  Configuration=Y (grounded)  NominalVoltage=[  Vabc=V_846_848*Vnom  Vabcp=[1.031 1.029 1.031]*sqrt(3)*Vnom  NominalFrequency=Frequency  UnbalancedPower=on  ActivePower=10e3  InductivePower=100  CapacitivePower=100  Pabc=Pa_846_848/2  QLabc=Pp_846_848/2  QCabc=Pn_846_848  Pabcp=[16 20 110]*1e3/2  QLabcp=[8 10 55]*1e3/2  QCabcp=[0 0 0]  Measurements=None  LoadType=constant PQ
      settings: SourceProductName=Simscape Electrical
      settings: AttributesFormatString=|
      | P= %<Pabc> W
      | Ql=%<QLabc> var
      | Qc=%<QCabc> var
  846-848 : powerlib/Elements/Distributed Parameters Line  Phases=3  Frequency=Frequency  Resistance=R_301  Inductance=L_301  Capacitance=C_301  Length=530*ft2km  x1=[535.070490121194 23931.5919189507 24208.9096649864;376.991118430775 376.991118430775 376.991118430775;-1.57116441842435 0.179521459636426 1.73136124814262]  x2=[535.726232674053 23935.0277330353 24213.0903489725;376.991118430775 376.991118430775 376.991118430775;-1.57136719456717 0.179154221564 1.73099838237163]  x3=[2.30674622159686 83.8715617487995 75.6598347764726;376.991118430775 376.991118430775 376.991118430775;-2.34643927784914 -0.467753379894094 0.997042978593791]  x4=[1.68367020204167 88.30646914241 79.56946272729;376.991118430775 376.991118430775 376.991118430775;0.287811005753666 0.788784613697999 2.42160577803868]  x5=7.30864815415796e-07  V1=ones(3,3)  V2=ones(3,3)  I1=ones(3,3)  I2=ones(3,3)  nHarmo=1  Measurements=None
      settings: SourceProductName=Simscape Electrical
  848 : powerlib/Measurements/Three-Phase V-I Measurement  VoltageMeasurement=phase-to-ground  SetLabelV=on  LabelV=Vabc_848  Vpu=on  VpuLL=off  CurrentMeasurement=yes  SetLabelI=on  LabelI=Iabc_848  Ipu=on  Pbase=100e6  Vbase=Vnom_ph_ph  OutputType=Magnitude-Angle  PhasorSimulation=on  PSBequivalent=0
      settings: SourceProductName=Simscape Electrical
  848 D-PQ : powerlib/Elements/Three-Phase Series RLC Load  LConnTagsString=A|B|C  Configuration=Delta  NominalVoltage=1000  Vabc=[1e3 1e3 1e3]  Vabcp=V_848*Vnom  NominalFrequency=Frequency  UnbalancedPower=on  ActivePower=[20 20 20]*1e3  InductivePower=[20 20 20]*1e3  CapacitivePower=100  Pabc=[10e3 9e3 11e3]  QLabc=[100 90 110]  QCabc=[100 90 110]  Pabcp=Pa_848  QLabcp=Pp_848  QCabcp=[0 0 0]  Measurements=Branch voltages and currents  LoadType=constant PQ
      settings: SourceProductName=Simscape Electrical
      settings: AttributesFormatString=|
      | P= %<Pabc> W
      | Ql=%<QLabc> var
      | Qc=%<QCabc> var
  848 D-Z : powerlib/Elements/Three-Phase Series RLC Load  LConnTagsString=A|B|C  Configuration=Delta  NominalVoltage=1000  Vabc=[1e3 1e3 1e3]  Vabcp="[1  1  1]*Vnom"  NominalFrequency=Frequency  UnbalancedPower=on  ActivePower=[20 20 20]*1e3  InductivePower=[20 20 20]*1e3  CapacitivePower=100  Pabc=[10e3 9e3 11e3]  QLabc=[100 90 110]  QCabc=[100 90 110]  Pabcp=[0 0 0]  QLabcp=[0 0 0]  QCabcp=Pn_848  Measurements=None  LoadType=constant Z
      settings: SourceProductName=Simscape Electrical
      settings: AttributesFormatString=|
      | P= %<Pabc> W
      | Ql=%<QLabc> var
      | Qc=%<QCabc> var
  848 Y-PQ : powerlib/Elements/Three-Phase Series RLC Load  LConnTagsString=A|B|C  Configuration=Y (grounded)  NominalVoltage=[  Vabc=V_846_848*Vnom  Vabcp=[1.031 1.029 1.031]*sqrt(3)*Vnom  NominalFrequency=Frequency  UnbalancedPower=on  ActivePower=10e3  InductivePower=100  CapacitivePower=100  Pabc=Pa_846_848/2  QLabc=Pp_846_848/2  QCabc=Pn_846_848  Pabcp=[16 20 110]*1e3/2  QLabcp=[8 10 55]*1e3/2  QCabcp=[0 0 0]  Measurements=None  LoadType=constant PQ
      settings: SourceProductName=Simscape Electrical
      settings: AttributesFormatString=|
      | P= %<Pabc> W
      | Ql=%<QLabc> var
      | Qc=%<QCabc> var
  850-816 : powerlib/Elements/Distributed Parameters Line  Phases=3  Frequency=Frequency  Resistance=R_301  Inductance=L_301  Capacitance=C_301  Length=310*ft2km  x1=[669.74621388492 24884.491056861 25124.8873333344;376.991118430775 376.991118430775 376.991118430775;-1.48270028181755 0.2401551161165 1.79952627773342]  x2=[669.297297756189 24878.5341192423 25120.2778264531;376.991118430775 376.991118430775 376.991118430775;-1.48601310209674 0.239952940684182 1.79927033881836]  x3=[10.6350315787157 19.7155932208958 31.0273020049027;376.991118430775 376.991118430775 376.991118430775;2.23983313205043 -1.14827391854565 0.149705684971895]  x4=[11.8830570336861 142.61168048345 128.187928121865;376.991118430775 376.991118430775 376.991118430775;-0.969511454617836 0.376360649041142 2.04303242710947]  x5=4.27486967507352e-07  V1=ones(3,3)  V2=ones(3,3)  I1=ones(3,3)  I2=ones(3,3)  nHarmo=1  Measurements=None
      settings: SourceProductName=Simscape Electrical
  852-832 : powerlib/Elements/Distributed Parameters Line  Phases=3  Frequency=Frequency  Resistance=R_301  Inductance=L_301  Capacitance=C_301  Length=10*ft2km  x1=[544.312287492488 23962.3241506796 24226.0097348477;376.991118430775 376.991118430775 376.991118430775;-1.57107506069415 0.191572562186321 1.7441306785241]  x2=[544.297192227652 23962.1985609162 24225.8886557252;376.991118430775 376.991118430775 376.991118430775;-1.57108853582541 0.191565398813415 1.74412250241144]  x3=[2.0451015642175 34.2046511338291 32.4638762615749;376.991118430775 376.991118430775 376.991118430775;1.09282641125666 -0.857965650826235 0.275869213477784]  x4=[3.14853201289675 126.050175505236 118.775868211036;376.991118430775 376.991118430775 376.991118430775;-1.87431844341811 0.429113210012534 2.019475569581]  x5=1.37899021776565e-08  V1=ones(3,3)  V2=ones(3,3)  I1=ones(3,3)  I2=ones(3,3)  nHarmo=1  Measurements=None
      settings: SourceProductName=Simscape Electrical
  854 Y-PQ : powerlib/Elements/Series RLC Load  LConnTagsString=a  RConnTagsString=__new0  NominalVoltage=V_854_856*Vnom  NominalFrequency=Frequency  ActivePower=Pa_854_856/2  InductivePower=Pp_854_856/2  CapacitivePower=Pn_854_856  Setx0=off  InitialVoltage=0  SetiL0=off  InitialCurrent=0  Measurements=None  LoadType=constant PQ
      settings: SourceProductName=Simscape Electrical
      settings: AttributesFormatString=|
      | P=%<ActivePower> W
      | Ql=%<InductivePower> var
      | Qc=%<CapacitivePower> var
  854-852 : powerlib/Elements/Distributed Parameters Line  Phases=3  Frequency=Frequency  Resistance=R_301  Inductance=L_301  Capacitance=C_301  Length=36830*ft2km  x1=[600.415344439585 24430.2182967214 24679.9493391831;376.991118430775 376.991118430775 376.991118430775;-1.54505377262824 0.202116204163532 1.75855303215963]  x2=[544.312287492488 23962.3241506796 24226.0097348477;376.991118430775 376.991118430775 376.991118430775;-1.59021656600906 0.175972515488602 1.72877526687479]  x3=[1.9844464227648 33.3694405463501 31.2384349468516;376.991118430775 376.991118430775 376.991118430775;1.05260156125433 -0.843535884234991 0.284210540813551]  x4=[3.11830583749387 123.340307988547 116.705348459943;376.991118430775 376.991118430775 376.991118430775;-1.89370372795784 0.414631277754311 2.00507902016042]  x5=5.0788209720309e-05  V1=ones(3,3)  V2=ones(3,3)  I1=ones(3,3)  I2=ones(3,3)  nHarmo=1  Measurements=None
      settings: SourceProductName=Simscape Electrical
  854-856 : powerlib/Elements/Distributed Parameters Line  Phases=1  Frequency=Frequency  Resistance=R_303(2,2)  Inductance=L_303(2,2)  Capacitance=C_303(2,2)  Length=23330*ft2km  x1=[20406.7886977255;376.991118430775;-2.20385345559487]  x2=[20404.9358015447;376.991118430775;-2.20397259567372]  x3=[33.6868271192158;376.991118430775;-2.21213224973626]  x4=[34.075157038624;376.991118430775;-2.20685151434764]  x5=2.9363349960162e-05  V1=ones(3,3)  V2=ones(3,3)  I1=ones(3,3)  I2=ones(3,3)  nHarmo=1  Measurements=None
      settings: SourceProductName=Simscape Electrical
  856 Y-PQ : powerlib/Elements/Series RLC Load  LConnTagsString=a  RConnTagsString=__new0  NominalVoltage=V_854_856*Vnom  NominalFrequency=Frequency  ActivePower=Pa_854_856/2  InductivePower=Pp_854_856/2  CapacitivePower=Pn_854_856  Setx0=off  InitialVoltage=0  SetiL0=off  InitialCurrent=0  Measurements=None  LoadType=constant PQ
      settings: SourceProductName=Simscape Electrical
      settings: AttributesFormatString=|
      | P=%<ActivePower> W
      | Ql=%<InductivePower> var
      | Qc=%<CapacitivePower> var
  858 : powerlib/Measurements/Three-Phase V-I Measurement  VoltageMeasurement=phase-to-ground  SetLabelV=on  LabelV=Vabc_858  Vpu=on  VpuLL=off  CurrentMeasurement=yes  SetLabelI=on  LabelI=Iabc_858  Ipu=on  Pbase=100e6  Vbase=Vnom_ph_ph  OutputType=Magnitude-Angle  PhasorSimulation=on  PSBequivalent=0
      settings: SourceProductName=Simscape Electrical
  858 D-PQ : powerlib/Elements/Three-Phase Series RLC Load  LConnTagsString=A|B|C  Configuration=Delta  NominalVoltage=[  Vabc=[1.017 1.025 1.02]*sqrt(3)*Vnom  Vabcp=V_858_834*Vnom  NominalFrequency=Frequency  UnbalancedPower=on  ActivePower=10e3  InductivePower=100  CapacitivePower=100  Pabc=[0 30 25]*1e3/2  QLabc=[0 15 14]*1e3/2  QCabc=[0 0 0]  Pabcp=Pa_858_834/2  QLabcp=Pp_858_834/2  QCabcp=Pn_858_834  Measurements=None  LoadType=constant PQ
      settings: SourceProductName=Simscape Electrical
      settings: AttributesFormatString=|
      | P= %<Pabc> W
      | Ql=%<QLabc> var
      | Qc=%<QCabc> var
  858 D-Z : powerlib/Elements/Three-Phase Series RLC Load  LConnTagsString=A|B|C  Configuration=Delta  NominalVoltage=[  Vabc=[1.017 1.025 1.02]*sqrt(3)*Vnom  Vabcp=V_832_858*Vnom  NominalFrequency=Frequency  UnbalancedPower=on  ActivePower=10e3  InductivePower=100  CapacitivePower=100  Pabc=[0 30 25]*1e3/2  QLabc=[0 15 14]*1e3/2  QCabc=[0 0 0]  Pabcp=Pa_832_858/2  QLabcp=Pp_832_858/2  QCabcp=Pn_832_858  Measurements=None  LoadType=constant Z
      settings: SourceProductName=Simscape Electrical
      settings: AttributesFormatString=|
      | P= %<Pabc> W
      | Ql=%<QLabc> var
      | Qc=%<QCabc> var
  858 Y-PQ : powerlib/Elements/Series RLC Load  LConnTagsString=a  RConnTagsString=__new0  NominalVoltage=1.034*Vnom  NominalFrequency=Frequency  ActivePower=Pa_858_864/2  InductivePower=Pp_858_864/2  CapacitivePower=Pn_858_864  Setx0=off  InitialVoltage=0  SetiL0=off  InitialCurrent=0  Measurements=None  LoadType=constant PQ
      settings: SourceProductName=Simscape Electrical
      settings: AttributesFormatString=|
      | P=%<ActivePower> W
      | Ql=%<InductivePower> var
      | Qc=%<CapacitivePower> var
  858-834 : powerlib/Elements/Distributed Parameters Line  Phases=3  Frequency=Frequency  Resistance=R_301  Inductance=L_301  Capacitance=C_301  Length=5830*ft2km  x1=[538.916079582122 23936.381353331 24203.4007325891;376.991118430775 376.991118430775 376.991118430775;-1.57575865553446 0.185474774270013 1.73766511633479]  x2=[532.488097890623 23907.9048332495 24179.347575776;376.991118430775 376.991118430775 376.991118430775;-1.57668635941168 0.181152075194233 1.73288360391624]  x3=[1.3322402193524 53.7985853583723 48.2778369020834;376.991118430775 376.991118430775 376.991118430775;0.514549779921959 -0.65524486646589 0.650059790973734]  x4=[2.16506190399758 110.228691971368 103.665767209341;376.991118430775 376.991118430775 376.991118430775;-2.14052175083063 0.553090897851426 2.15827631696394]  x5=8.03951296957376e-06  V1=ones(3,3)  V2=ones(3,3)  I1=ones(3,3)  I2=ones(3,3)  nHarmo=1  Measurements=None
      settings: SourceProductName=Simscape Electrical
  858-864 : powerlib/Elements/Distributed Parameters Line  Phases=1  Frequency=Frequency  Resistance=R_302(1,1)  Inductance=L_302(1,1)  Capacitance=C_302(1,1)  Length=1620*ft2km  x1=[19061.7942628737;376.991118430775;-0.112504967132919]  x2=[19061.7061369417;376.991118430775;-0.112505642938732]  x3=[32.0263026700578;376.991118430775;-0.111930141076138]  x4=[32.1985862565088;376.991118430775;-0.113844277485216]  x5=2.03894671819385e-06  V1=ones(3,3)  V2=ones(3,3)  I1=ones(3,3)  I2=ones(3,3)  nHarmo=1  Measurements=None
      settings: SourceProductName=Simscape Electrical
  860 : powerlib/Measurements/Three-Phase V-I Measurement  VoltageMeasurement=phase-to-ground  SetLabelV=on  LabelV=Vabc_860  Vpu=on  VpuLL=off  CurrentMeasurement=yes  SetLabelI=on  LabelI=Iabc_860  Ipu=on  Pbase=100e6  Vbase=Vnom_ph_ph  OutputType=Magnitude-Angle  PhasorSimulation=on  PSBequivalent=0
      settings: SourceProductName=Simscape Electrical
  860 D-PQ : powerlib/Elements/Three-Phase Series RLC Load  LConnTagsString=A|B|C  Configuration=Delta  NominalVoltage=[  Vabc=[1.017 1.025 1.02]*sqrt(3)*Vnom  Vabcp=V_860_836*Vnom  NominalFrequency=Frequency  UnbalancedPower=on  ActivePower=10e3  InductivePower=100  CapacitivePower=100  Pabc=[0 30 25]*1e3/2  QLabc=[0 15 14]*1e3/2  QCabc=[0 0 0]  Pabcp=Pa_860_836/2  QLabcp=Pp_860_836/2  QCabcp=Pn_860_836  Measurements=None  LoadType=constant PQ
      settings: SourceProductName=Simscape Electrical
      settings: AttributesFormatString=|
      | P= %<Pabc> W
      | Ql=%<QLabc> var
      | Qc=%<QCabc> var
  860 D-Z : powerlib/Elements/Three-Phase Series RLC Load  LConnTagsString=A|B|C  Configuration=Delta  NominalVoltage=[  Vabc=[1.017 1.025 1.02]*sqrt(3)*Vnom  Vabcp=V_834_860*Vnom  NominalFrequency=Frequency  UnbalancedPower=on  ActivePower=10e3  InductivePower=100  CapacitivePower=100  Pabc=[0 30 25]*1e3/2  QLabc=[0 15 14]*1e3/2  QCabc=[0 0 0]  Pabcp=Pa_834_860/2  QLabcp=Pp_834_860/2  QCabcp=Pn_834_860  Measurements=None  LoadType=constant Z
      settings: SourceProductName=Simscape Electrical
      settings: AttributesFormatString=|
      | P= %<Pabc> W
      | Ql=%<QLabc> var
      | Qc=%<QCabc> var
  860 Y-PQ : powerlib/Elements/Three-Phase Series RLC Load  LConnTagsString=A|B|C  Configuration=Y (grounded)  NominalVoltage=[  Vabc=V_860*Vnom  Vabcp=[1.031 1.029 1.031]*sqrt(3)*Vnom  NominalFrequency=Frequency  UnbalancedPower=on  ActivePower=10e3  InductivePower=100  CapacitivePower=100  Pabc=Pa_860  QLabc=Pp_860  QCabc=Pn_860  Pabcp=[16 20 110]*1e3/2  QLabcp=[8 10 55]*1e3/2  QCabcp=[0 0 0]  Measurements=None  LoadType=constant PQ
      settings: SourceProductName=Simscape Electrical
      settings: AttributesFormatString=|
      | P= %<Pabc> W
      | Ql=%<QLabc> var
      | Qc=%<QCabc> var
  860-836 : powerlib/Elements/Distributed Parameters Line  Phases=3  Frequency=Frequency  Resistance=R_301  Inductance=L_301  Capacitance=C_301  Length=2680*ft2km  x1=[529.898068973043 23898.4588495649 24170.0388321035;376.991118430775 376.991118430775 376.991118430775;-1.57508876728632 0.182546737459766 1.73418444772525]  x2=[526.843358587077 23892.7809998017 24164.7359964069;376.991118430775 376.991118430775 376.991118430775;-1.5740352997078 0.18250218138139 1.73424546111815]  x3=[1.5527482586932 63.5253292593436 54.6372337900891;376.991118430775 376.991118430775 376.991118430775;0.243311241443216 0.204981473863063 1.80565667873082]  x4=[2.1489415015772 75.4018639160811 62.7864228798159;376.991118430775 376.991118430775 376.991118430775;-2.35135466427602 0.162558445723816 1.67101328863283]  x5=3.69569378361195e-06  V1=ones(3,3)  V2=ones(3,3)  I1=ones(3,3)  I2=ones(3,3)  nHarmo=1  Measurements=None
      settings: SourceProductName=Simscape Electrical
  862 Y-PQ : powerlib/Elements/Series RLC Load  LConnTagsString=a  RConnTagsString=__new0  NominalVoltage=V_862_838*Vnom  NominalFrequency=Frequency  ActivePower=Pa_862_838/2  InductivePower=Pp_862_838/2  CapacitivePower=Pn_862_838  Setx0=off  InitialVoltage=0  SetiL0=off  InitialCurrent=0  Measurements=None  LoadType=constant PQ
      settings: SourceProductName=Simscape Electrical
      settings: AttributesFormatString=|
      | P=%<ActivePower> W
      | Ql=%<InductivePower> var
      | Qc=%<CapacitivePower> var
  862-838 : powerlib/Elements/Distributed Parameters Line  Phases=1  Frequency=Frequency  Resistance=R_304(2,2)  Inductance=L_304(2,2)  Capacitance=C_304(2,2)  Length=4860*ft2km  x1=[19984.3731061187;376.991118430775;-2.23186275136805]  x2=[19981.3282964726;376.991118430775;-2.23189340811562]  x3=[33.6649144176445;376.991118430775;-2.21528457460766]  x4=[36.2132789010856;376.991118430775;-2.24951705550692]  x5=6.08033278760362e-06  V1=ones(3,3)  V2=ones(3,3)  I1=ones(3,3)  I2=ones(3,3)  nHarmo=1  Measurements=None
      settings: SourceProductName=Simscape Electrical
  864 Y-PQ : powerlib/Elements/Series RLC Load  LConnTagsString=a  RConnTagsString=__new0  NominalVoltage=1.034*Vnom  NominalFrequency=Frequency  ActivePower=2e3/2  InductivePower=1e3/2  CapacitivePower=0  Setx0=off  InitialVoltage=0  SetiL0=off  InitialCurrent=0  Measurements=None  LoadType=constant PQ
      settings: SourceProductName=Simscape Electrical
      settings: AttributesFormatString=|
      | P=%<ActivePower> W
      | Ql=%<InductivePower> var
      | Qc=%<CapacitivePower> var
  888-890 : powerlib/Elements/Distributed Parameters Line  Phases=3  Frequency=Frequency  Resistance=R_300  Inductance=L_300  Capacitance=C_300  Length=10560*ft2km  x1=[258.824665684925 3850.67039835961 3891.13941195574;376.991118430775 376.991118430775 376.991118430775;2.16140852765149 0.159562565428488 1.71422558272713]  x2=[277.437082415887 3524.08362530415 3548.14342354217;376.991118430775 376.991118430775 376.991118430775;2.2028595426639 0.148082617443792 1.69508711329456]  x3=[4.2334583346631 111.19292312888 114.001682451802;376.991118430775 376.991118430775 376.991118430775;1.81336554107905 2.78094155494843 -1.95072583089264]  x4=[47.2489946102347 130.794318211806 130.408515234695;376.991118430775 376.991118430775 376.991118430775;1.23328833703807 -0.278160480236052 1.26027294844431]  x5=1.41710191462344e-05  V1=ones(3,3)  V2=ones(3,3)  I1=ones(3,3)  I2=ones(3,3)  nHarmo=1  Measurements=None
      settings: SourceProductName=Simscape Electrical
  890 : powerlib/Measurements/Three-Phase V-I Measurement  VoltageMeasurement=phase-to-ground  SetLabelV=on  LabelV=Vabc_890  Vpu=on  VpuLL=off  CurrentMeasurement=yes  SetLabelI=on  LabelI=Iabc_890  Ipu=on  Pbase=100e6  Vbase=Vnom1_ph_ph  OutputType=Magnitude-Angle  PhasorSimulation=on  PSBequivalent=0
      settings: SourceProductName=Simscape Electrical
  890 D-I : powerlib/Elements/Three-Phase Series RLC Load  LConnTagsString=A|B|C  Configuration=Delta  NominalVoltage=1000  Vabc=[1e3 1e3 1e3]  Vabcp=V_890*Vnom1  NominalFrequency=Frequency  UnbalancedPower=on  ActivePower=10e3  InductivePower=100  CapacitivePower=100  Pabc=[10e3 9e3 11e3]  QLabc=[100 90 110]  QCabc=[100 90 110]  Pabcp=Pa_890  QLabcp=Pp_890  QCabcp=Pn_890  Measurements=None  LoadType=constant I
      settings: SourceProductName=Simscape Electrical
  Ground{,1..5,8..15} (14 alike) : powerlib/Elements/Ground  LConnTagsString=a
      settings: SourceProductName=Simscape Electrical
  Load Flow Bus : powerlib/Measurements/Load Flow Bus  LConnTagsString=a|b|c  RConnTagsString=a|b|c  Phases=ABC  Connectors=on both sides  ID=800  Vbase=Vnom  Vref="[1.05  1.05  1.05]"  Vangle="[0  -120  120]"  VLF=1  VLFb=1  VLFc=1  angleLF=0  angleLFb=0  angleLFc=0
      settings: AttributesFormatString=%<ID>  SourceProductName=Simscape Electrical
  Load Flow Bus1 : powerlib/Measurements/Load Flow Bus  LConnTagsString=a|b|c  RConnTagsString=a|b|c  Phases=ABC  Connectors=on both sides  ID=802  Vbase=Vnom  Vref=[1.0475 1.0484 1.0484]  Vangle=[-0.05 -120.07 119.95]  VLF=1  VLFb=1  VLFc=1  angleLF=0  angleLFb=0  angleLFc=0
      settings: AttributesFormatString=%<ID>  SourceProductName=Simscape Electrical
  Load Flow Bus10 : powerlib/Measurements/Load Flow Bus  LConnTagsString=a  Phases=B  Connectors=on one side  ID=826  Vbase=Vnom  Vref=1.0156  Vangle=-122.94  VLF=1  VLFb=1  VLFc=1  angleLF=0  angleLFb=0  angleLFc=0
      settings: AttributesFormatString=%<ID>  SourceProductName=Simscape Electrical
  Load Flow Bus11 : powerlib/Measurements/Load Flow Bus  LConnTagsString=a  RConnTagsString=a  Phases=A  Connectors=on both sides  ID=818  Vbase=Vnom  Vref=1.0163  Vangle=-2.27  VLF=1  VLFb=1  VLFc=1  angleLF=0  angleLFb=0  angleLFc=0
      settings: AttributesFormatString=%<ID>  SourceProductName=Simscape Electrical
  Load Flow Bus12 : powerlib/Measurements/Load Flow Bus  LConnTagsString=a  RConnTagsString=a  Phases=A  Connectors=on both sides  ID=820  Vbase=Vnom  Vref=0.9926  Vangle=-2.32  VLF=1  VLFb=1  VLFc=1  angleLF=0  angleLFb=0  angleLFc=0
      settings: AttributesFormatString=%<ID>  SourceProductName=Simscape Electrical
  Load Flow Bus13 : powerlib/Measurements/Load Flow Bus  LConnTagsString=a  Phases=A  Connectors=on one side  ID=822  Vbase=Vnom  Vref=0.9895  Vangle=-2.33  VLF=1  VLFb=1  VLFc=1  angleLF=0  angleLFb=0  angleLFc=0
      settings: AttributesFormatString=%<ID>  SourceProductName=Simscape Electrical
  Load Flow Bus14 : powerlib/Measurements/Load Flow Bus  LConnTagsString=a|b|c  RConnTagsString=a|b|c  Phases=ABC  Connectors=on both sides  ID=828  Vbase=Vnom  Vref=[1.0074 1.0151 1.0109]  Vangle=[-2.38 -122.95 117.75]  VLF=1  VLFb=1  VLFc=1  angleLF=0  angleLFb=0  angleLFc=0
      settings: AttributesFormatString=%<ID>  SourceProductName=Simscape Electrical
  Load Flow Bus15 : powerlib/Measurements/Load Flow Bus  LConnTagsString=a|b|c  RConnTagsString=a|b|c  Phases=ABC  Connectors=on both sides  ID=830  Vbase=Vnom  Vref=[0.9894 0.9982 0.9938]  Vangle=[-2.63 -123.39 117.25]  VLF=1  VLFb=1  VLFc=1  angleLF=0  angleLFb=0  angleLFc=0
      settings: AttributesFormatString=%<ID>  SourceProductName=Simscape Electrical
  Load Flow Bus16 : powerlib/Measurements/Load Flow Bus  LConnTagsString=a|b|c  RConnTagsString=a|b|c  Phases=ABC  Connectors=on both sides  ID=854  Vbase=Vnom  Vref=[0.989 0.9978 0.9934]  Vangle=[-2.64 -123.4 117.24]  VLF=1  VLFb=1  VLFc=1  angleLF=0  angleLFb=0  angleLFc=0
      settings: AttributesFormatString=%<ID>  SourceProductName=Simscape Electrical
  Load Flow Bus17 : powerlib/Measurements/Load Flow Bus  LConnTagsString=a  Phases=B  Connectors=on one side  ID=856  Vbase=Vnom  Vref=0.9977  Vangle=-123.41  VLF=1  VLFb=1  VLFc=1  angleLF=0  angleLFb=0  angleLFc=0
      settings: AttributesFormatString=%<ID>  SourceProductName=Simscape Electrical
  Load Flow Bus18 : powerlib/Measurements/Load Flow Bus  LConnTagsString=a|b|c  RConnTagsString=a|b|c  Phases=ABC  Connectors=on both sides  ID=852  Vbase=Vnom  Vref=[0.9581 0.968 0.9637]  Vangle=[-3.11 -124.18 116.33]  VLF=1  VLFb=1  VLFc=1  angleLF=0  angleLFb=0  angleLFc=0
      settings: AttributesFormatString=%<ID>  SourceProductName=Simscape Electrical
  Load Flow Bus19 : powerlib/Measurements/Load Flow Bus  LConnTagsString=a|b|c  RConnTagsString=a|b|c  Phases=ABC  Connectors=on both sides  ID=832  Vbase=Vnom  Vref=[1.0359 1.0345 1.036]  Vangle=[-3.11 -124.18 116.33]  VLF=1  VLFb=1  VLFc=1  angleLF=0  angleLFb=0  angleLFc=0
      settings: AttributesFormatString=%<ID>  SourceProductName=Simscape Electrical
  Load Flow Bus2 : powerlib/Measurements/Load Flow Bus  LConnTagsString=a|b|c  RConnTagsString=a|b|c  Phases=ABC  Connectors=on both sides  ID=806  Vbase=Vnom  Vref=[1.0457 1.0474 1.0474]  Vangle=[-0.08 -120.11 119.92]  VLF=1  VLFb=1  VLFc=1  angleLF=0  angleLFb=0  angleLFc=0
      settings: AttributesFormatString=%<ID>  SourceProductName=Simscape Electrical
  Load Flow Bus20 : powerlib/Measurements/Load Flow Bus  LConnTagsString=a|b|c  RConnTagsString=a|b|c  Phases=ABC  Connectors=on both sides  ID=888  Vbase=Vnom1  Vref=[0.9996 0.9983 1]  Vangle=[-4.64 -125.73 114.82]  VLF=1  VLFb=1  VLFc=1  angleLF=0  angleLFb=0  angleLFc=0
      settings: AttributesFormatString=%<ID>  SourceProductName=Simscape Electrical
  Load Flow Bus21 : powerlib/Measurements/Load Flow Bus  LConnTagsString=a|b|c  RConnTagsString=a|b|c  Phases=ABC  Connectors=on both sides  ID=890  Vbase=Vnom1  Vref=[0.9167 0.9235 0.9177]  Vangle=[-5.19 -126.78 113.98]  VLF=1  VLFb=1  VLFc=1  angleLF=0  angleLFb=0  angleLFc=0
      settings: AttributesFormatString=%<ID>  SourceProductName=Simscape Electrical
  Load Flow Bus22 : powerlib/Measurements/Load Flow Bus  LConnTagsString=a|b|c  RConnTagsString=a|b|c  Phases=ABC  Connectors=on both sides  ID=858  Vbase=Vnom  Vref=[1.0336 1.0322 1.0338]  Vangle=[-3.17 -124.28 116.22]  VLF=1  VLFb=1  VLFc=1  angleLF=0  angleLFb=0  angleLFc=0
      settings: AttributesFormatString=%<ID>  SourceProductName=Simscape Electrical
  Load Flow Bus23 : powerlib/Measurements/Load Flow Bus  LConnTagsString=a  Phases=A  Connectors=on one side  ID=864  Vbase=Vnom  Vref=1.0336  Vangle=-3.17  VLF=1  VLFb=1  VLFc=1  angleLF=0  angleLFb=0  angleLFc=0
      settings: AttributesFormatString=%<ID>  SourceProductName=Simscape Electrical
  Load Flow Bus24 : powerlib/Measurements/Load Flow Bus  LConnTagsString=a|b|c  RConnTagsString=a|b|c  Phases=ABC  Connectors=on both sides  ID=834  Vbase=Vnom  Vref=[1.0309 1.0295 1.0313]  Vangle=[-3.24 -124.39 116.09]  VLF=1  VLFb=1  VLFc=1  angleLF=0  angleLFb=0  angleLFc=0
      settings: AttributesFormatString=%<ID>  SourceProductName=Simscape Electrical
  Load Flow Bus25 : powerlib/Measurements/Load Flow Bus  LConnTagsString=a|b|c  RConnTagsString=a|b|c  Phases=ABC  Connectors=on both sides  ID=860  Vbase=Vnom  Vref=[1.0305 1.0291 1.031]  Vangle=[-3.24 -124.39 116.09]  VLF=1  VLFb=1  VLFc=1  angleLF=0  angleLFb=0  angleLFc=0
      settings: AttributesFormatString=%<ID>  SourceProductName=Simscape Electrical
  Load Flow Bus26 : powerlib/Measurements/Load Flow Bus  LConnTagsString=a|b|c  RConnTagsString=a|b|c  Phases=ABC  Connectors=on both sides  ID=836  Vbase=Vnom  Vref=[1.0303 1.0287 1.0308]  Vangle=[-3.23 -124.39 116.09]  VLF=1  VLFb=1  VLFc=1  angleLF=0  angleLFb=0  angleLFc=0
      settings: AttributesFormatString=%<ID>  SourceProductName=Simscape Electrical
  Load Flow Bus27 : powerlib/Measurements/Load Flow Bus  LConnTagsString=a|b|c  RConnTagsString=a|b|c  Phases=ABC  Connectors=on both sides  ID=840  Vbase=Vnom  Vref=[1.0303 1.0287 1.0308]  Vangle=[-3.23 -124.39 116.09]  VLF=1  VLFb=1  VLFc=1  angleLF=0  angleLFb=0  angleLFc=0
      settings: AttributesFormatString=%<ID>  SourceProductName=Simscape Electrical
  Load Flow Bus29 : powerlib/Measurements/Load Flow Bus  LConnTagsString=a  Phases=B  Connectors=on one side  ID=838  Vbase=Vnom  Vref=1.0285  Vangle=-124.39  VLF=1  VLFb=1  VLFc=1  angleLF=0  angleLFb=0  angleLFc=0
      settings: AttributesFormatString=%<ID>  SourceProductName=Simscape Electrical
  Load Flow Bus3 : powerlib/Measurements/Load Flow Bus  LConnTagsString=a|b|c  RConnTagsString=a|b|c  Phases=ABC  Connectors=on both sides  ID=808  Vbase=Vnom  Vref=[1.0136 1.0296 1.0289]  Vangle=[-0.75 -120.95 119.3]  VLF=1  VLFb=1  VLFc=1  angleLF=0  angleLFb=0  angleLFc=0
      settings: AttributesFormatString=%<ID>  SourceProductName=Simscape Electrical
  Load Flow Bus30 : powerlib/Measurements/Load Flow Bus  LConnTagsString=a|b|c  RConnTagsString=a|b|c  Phases=ABC  Connectors=on both sides  ID=842  Vbase=Vnom  Vref=[1.0309 1.0294 1.0313]  Vangle=[-3.25 -124.39 116.09]  VLF=1  VLFb=1  VLFc=1  angleLF=0  angleLFb=0  angleLFc=0
      settings: AttributesFormatString=%<ID>  SourceProductName=Simscape Electrical
  Load Flow Bus31 : powerlib/Measurements/Load Flow Bus  LConnTagsString=a|b|c  RConnTagsString=a|b|c  Phases=ABC  Connectors=on both sides  ID=844  Vbase=Vnom  Vref=[1.0307 1.0291 1.0311]  Vangle=[-3.27 -124.42 116.06]  VLF=1  VLFb=1  VLFc=1  angleLF=0  angleLFb=0  angleLFc=0
      settings: AttributesFormatString=%<ID>  SourceProductName=Simscape Electrical
  Load Flow Bus32 : powerlib/Measurements/Load Flow Bus  LConnTagsString=a|b|c  RConnTagsString=a|b|c  Phases=ABC  Connectors=on both sides  ID=846  Vbase=Vnom  Vref=[1.0309 1.0291 1.0313]  Vangle=[-3.32 -124.46 116.01]  VLF=1  VLFb=1  VLFc=1  angleLF=0  angleLFb=0  angleLFc=0
      settings: AttributesFormatString=%<ID>  SourceProductName=Simscape Electrical
  Load Flow Bus33 : powerlib/Measurements/Load Flow Bus  LConnTagsString=a|b|c  RConnTagsString=a|b|c  Phases=ABC  Connectors=on both sides  ID=848  Vbase=Vnom  Vref=[1.031 1.0291 1.0314]  Vangle=[-3.32 -124.47 116]  VLF=1  VLFb=1  VLFc=1  angleLF=0  angleLFb=0  angleLFc=0
      settings: AttributesFormatString=%<ID>  SourceProductName=Simscape Electrical
  Load Flow Bus34 : powerlib/Measurements/Load Flow Bus  LConnTagsString=a  Phases=A  Connectors=on one side  ID=open862  Vbase=Vnom  Vref=1.0303  Vangle=-3.23  VLF=1  VLFb=1  VLFc=1  angleLF=0  angleLFb=0  angleLFc=0
      settings: AttributesFormatString=%<ID>  SourceProductName=Simscape Electrical
  Load Flow Bus35 : powerlib/Measurements/Load Flow Bus  LConnTagsString=a  Phases=C  Connectors=on one side  ID=open862  Vbase=Vnom  Vref=1.0308  Vangle=116.09  VLF=1  VLFb=1  VLFc=1  angleLF=0  angleLFb=0  angleLFc=0
      settings: AttributesFormatString=%<ID>  SourceProductName=Simscape Electrical
  Load Flow Bus36 : powerlib/Measurements/Load Flow Bus  LConnTagsString=a  RConnTagsString=a  Phases=B  Connectors=on both sides  ID=862  Vbase=Vnom  Vref=1.0287  Vangle=-124.39  VLF=1  VLFb=1  VLFc=1  angleLF=0  angleLFb=0  angleLFc=0
      settings: AttributesFormatString=%<ID>  SourceProductName=Simscape Electrical
  Load Flow Bus4 : powerlib/Measurements/Load Flow Bus  LConnTagsString=a|b|c  RConnTagsString=a|b|c  Phases=ABC  Connectors=on both sides  ID=812  Vbase=Vnom  Vref=[0.9763 1.01 1.0069]  Vangle=[-1.57 -121.92 118.59]  VLF=1  VLFb=1  VLFc=1  angleLF=0  angleLFb=0  angleLFc=0
      settings: AttributesFormatString=%<ID>  SourceProductName=Simscape Electrical
  Load Flow Bus5 : powerlib/Measurements/Load Flow Bus  LConnTagsString=a|b|c  RConnTagsString=a|b|c  Phases=ABC  Connectors=on both sides  ID=814  Vbase=Vnom  Vref=[0.9467 0.9945 0.9893]  Vangle=[-2.26 -122.7 118.01]  VLF=1  VLFb=1  VLFc=1  angleLF=0  angleLFb=0  angleLFc=0
      settings: AttributesFormatString=%<ID>  SourceProductName=Simscape Electrical
  Load Flow Bus6 : powerlib/Measurements/Load Flow Bus  LConnTagsString=a  Phases=B  Connectors=on one side  ID=810  Vbase=Vnom  Vref=1.0294  Vangle=-120.95  VLF=1  VLFb=1  VLFc=1  angleLF=0  angleLFb=0  angleLFc=0
      settings: AttributesFormatString=%<ID>  SourceProductName=Simscape Electrical
  Load Flow Bus7 : powerlib/Measurements/Load Flow Bus  LConnTagsString=a|b|c  RConnTagsString=a|b|c  Phases=ABC  Connectors=on both sides  ID=850  Vbase=Vnom  Vref=[1.0176 1.0255 1.0203]  Vangle=[-2.26 -122.7 118.01]  VLF=1  VLFb=1  VLFc=1  angleLF=0  angleLFb=0  angleLFc=0
      settings: AttributesFormatString=%<ID>  SourceProductName=Simscape Electrical
  Load Flow Bus8 : powerlib/Measurements/Load Flow Bus  LConnTagsString=a|b|c  RConnTagsString=a|b|c  Phases=ABC  Connectors=on both sides  ID=816  Vbase=Vnom  Vref=[1.0172 1.0253 1.02]  Vangle=[-2.26 -122.71 1.02]  VLF=1  VLFb=1  VLFc=1  angleLF=0  angleLFb=0  angleLFc=0
      settings: AttributesFormatString=%<ID>  SourceProductName=Simscape Electrical
  Load Flow Bus9 : powerlib/Measurements/Load Flow Bus  LConnTagsString=a|b|c  RConnTagsString=a|b|c  Phases=ABC  Connectors=on both sides  ID=824  Vbase=Vnom  Vref=[1.0082 1.0158 1.0116]  Vangle=[-2.37 -122.94 117.76]  VLF=1  VLFb=1  VLFc=1  angleLF=0  angleLFb=0  angleLFc=0
      settings: AttributesFormatString=%<ID>  SourceProductName=Simscape Electrical
  MultiStateImage : MultiStateImageBlock  ScaleMode=Fill  WebBlockId=177
  Power-Flow : Subsystem
      mask Display: disp('Power-Flow\nResults')
  XF-10 24.9kV / 4.16kV : powerlib/Elements/Three-Phase Transformer (Two Windings)  Winding1Connection=Yg  Winding2Connection=Yg  CoreType=Three single-phase transformers  SetSaturation=off  Hysteresis=off  DataFile='hysteresis'  SetInitialFlux=off  Measurements=None  UNITS=pu  NominalPower=[ 500e3 , 60 ]  Winding1=[ 24.9e3 , 0.019 , 0.0408 ]  Winding2=[ 4.16e3 , 0 , 0 ]  Rm=500  Lm=500  L0=0.5  Saturation=[ 0,0 ; 0.0024,1.2 ; 1.0,1.52 ]  InitialFluxes=[ 0.8 , -0.8 , 0.7 ]  BreakLoop=off  DiscreteSolver=Trapezoidal iterative  DataType=off  TransfoNumber=1
      settings: SourceProductName=Simscape Electrical
  powergui : powerlib/powergui  Priority=1  SimulationMode=Phasor  SampleTime=50e-6  frequency=60  Iterations=50  frequencyindice=60  Pbase=100e3  ErrMax=0.0001  UnitsV=kV  UnitsW=kW  buscounter=0  FunctionMessages=off  echomessages=off  EnableUseOfTLC=off  CurrentSourceSwitches=off  DisableSnubberDevices=off  DisableRonSwitches=off  DisableVfSwitches=off  DisplayEquations=off  AutomaticDiscreteSolvers=off  SolverType=Tustin/Backward Euler (TBE)  Interpol=off  ExternalGateDelay=off  methode=off  Ts=100  x0status=blocks  SPID=off  SwTol=0  HookPort=off  NonlinearTolerance=1e-4  nMaxIteration=100  ContinueOnMaxIteration=off  RestoreLinks=warning  ResistiveCurrentMeasurement=off  Frange=[0:2:500]  Ylog=off  Xlog=on  ShowGrid=off  save=off  variable=ZData  structure=0  ZoomFFT=on  StartTime=0.0  cycles=1  DisplayStyle=1  fundamental=60  FreqAxis=off  MaxFrequency=1000  frequencyindicesteady=1  RmsSteady=1  display=off
      settings: SourceProductName=Simscape Electrical
  connections:
  800 gen/RConn1 -- Load Flow Bus/LConn1
  800 gen/RConn2 -- Load Flow Bus/LConn2
  800 gen/RConn3 -- Load Flow Bus/LConn3
  800-802/RConn1 -- Load Flow Bus1/LConn1
  800-802/RConn2 -- Load Flow Bus1/LConn2
  800-802/RConn3 -- Load Flow Bus1/LConn3
  802/LConn1 -- Load Flow Bus1/RConn1
  802/LConn2 -- Load Flow Bus1/RConn2
  802/LConn3 -- Load Flow Bus1/RConn3
  802-806/LConn1 -- 802/RConn1 -- 802 Yg PQ/LConn1
  802-806/LConn2 -- 802/RConn2 -- 802 Yg PQ/LConn2
  802-806/LConn3 -- 802/RConn3 -- 802 Yg PQ/LConn3
  Load Flow Bus2/LConn1 -- 802-806/RConn1 -- 806 Yg PQ/LConn1
  Load Flow Bus2/LConn2 -- 802-806/RConn2 -- 806 Yg PQ/LConn2
  Load Flow Bus2/LConn3 -- 806 Yg PQ/LConn3 -- 802-806/RConn3
  808/LConn2 -- Load Flow Bus3/RConn2
  808/LConn3 -- Load Flow Bus3/RConn3
  Load Flow Bus3/LConn3 -- 806-808/RConn3
  Load Flow Bus3/LConn1 -- 806-808/RConn1
  Load Flow Bus3/LConn2 -- 806-808/RConn2
  808/LConn1 -- Load Flow Bus3/RConn1
  Load Flow Bus4/LConn3 -- 808-812/RConn3
  Load Flow Bus4/LConn1 -- 808-812/RConn1
  Load Flow Bus4/LConn2 -- 808-812/RConn2
  808-812/LConn1 -- 808/RConn1
  808-812/LConn2 -- 808 Y-I/LConn1 -- 808-810/LConn1 -- 808/RConn2
  808-812/LConn3 -- 808/RConn3
  Load Flow Bus5/LConn3 -- 812-814/RConn3
  Load Flow Bus5/LConn1 -- 812-814/RConn1
  Load Flow Bus5/LConn2 -- 812-814/RConn2
  Load Flow Bus7/LConn1 -- 814-850/RConn1
  Load Flow Bus7/LConn2 -- 814-850/RConn2
  Load Flow Bus7/LConn3 -- 814-850/RConn3
  816/LConn3 -- Load Flow Bus8/RConn3
  816/LConn1 -- Load Flow Bus8/RConn1
  816/LConn2 -- Load Flow Bus8/RConn2
  Load Flow Bus8/LConn2 -- 850-816/RConn2
  Load Flow Bus8/LConn3 -- 850-816/RConn3
  Load Flow Bus8/LConn1 -- 850-816/RConn1
  Load Flow Bus9/LConn2 -- 824 D-I/LConn2 -- 816-824/RConn2
  824/LConn1 -- Load Flow Bus9/RConn1
  Load Flow Bus9/LConn1 -- 824 D-I/LConn1 -- 816-824/RConn1
  824/LConn2 -- Load Flow Bus9/RConn2
  824/LConn3 -- Load Flow Bus9/RConn3
  Load Flow Bus9/LConn3 -- 824 D-I/LConn3 -- 816-824/RConn3
  816-824/LConn1 -- 816-818/LConn1 -- 816 D-I/LConn1 -- 816/RConn1
  816-824/LConn2 -- 816 D-I/LConn2 -- 816/RConn2
  816-824/LConn3 -- 816 D-I/LConn3 -- 816/RConn3
  824-828/LConn1 -- 824 Y-PQ/LConn1 -- 824/RConn1
  824-828/LConn2 -- 824 Y-PQ/LConn2 -- 824-826/LConn1 -- 824 Y-I/LConn1 -- 824/RConn2
  824-828/LConn3 -- 824 Y-PQ/LConn3 -- 824/RConn3
  818 Y-Z/LConn1 -- 818-820/LConn1 -- Load Flow Bus11/RConn1
  820 Y-PQ/LConn1 -- 820-822/LConn1 -- Load Flow Bus12/RConn1
  820 Y-Z/LConn1 -- 818-820/RConn1 -- Load Flow Bus12/LConn1
  822 Y-PQ/LConn1 -- Load Flow Bus13/LConn1 -- 820-822/RConn1
  828/LConn2 -- Load Flow Bus14/RConn2
  Load Flow Bus14/LConn3 -- 824-828/RConn3 -- 828 Y-PQ/LConn3
  828/LConn1 -- Load Flow Bus14/RConn1
  Load Flow Bus14/LConn1 -- 828 Y-PQ/LConn1 -- 824-828/RConn1
  828/LConn3 -- Load Flow Bus14/RConn3
  Load Flow Bus14/LConn2 -- 824-828/RConn2 -- 828 Y-PQ/LConn2
  830 Y-PQ/LConn1 -- Load Flow Bus15/LConn1 -- 828-830/RConn1
  830 Y-PQ/LConn2 -- Load Flow Bus15/LConn2 -- 828-830/RConn2
  830 Y-PQ/LConn3 -- Load Flow Bus15/LConn3 -- 828-830/RConn3
  828-830/LConn1 -- 828 Y-PQ1/LConn1 -- 828/RConn1
  828-830/LConn2 -- 828 Y-PQ1/LConn2 -- 828/RConn2
  828-830/LConn3 -- 828 Y-PQ1/LConn3 -- 828/RConn3
  Load Flow Bus16/LConn1 -- 830-854/RConn1
  Load Flow Bus16/LConn2 -- 830-854/RConn2
  Load Flow Bus16/LConn3 -- 830-854/RConn3
  Load Flow Bus18/LConn1 -- 854-852/RConn1
  Load Flow Bus18/LConn3 -- 854-852/RConn3
  Load Flow Bus18/LConn2 -- 854-852/RConn2
  Load Flow Bus19/LConn3 -- 852-832/RConn3
  Load Flow Bus19/LConn2 -- 852-832/RConn2
  832/LConn1 -- Load Flow Bus19/RConn1
  Load Flow Bus19/LConn1 -- 852-832/RConn1
  832/LConn2 -- Load Flow Bus19/RConn2
  832/LConn3 -- Load Flow Bus19/RConn3
  Load Flow Bus16/RConn2 -- 854-856/LConn1 -- 854 Y-PQ/LConn1 -- 854-852/LConn2
  Load Flow Bus16/RConn3 -- 854-852/LConn3
  Load Flow Bus16/RConn1 -- 854-852/LConn1
  890/LConn1 -- Load Flow Bus21/RConn1
  890/LConn2 -- Load Flow Bus21/RConn2
  Load Flow Bus21/LConn1 -- 888-890/RConn1
  Load Flow Bus21/LConn2 -- 888-890/RConn2
  890/LConn3 -- Load Flow Bus21/RConn3
  Load Flow Bus21/LConn3 -- 888-890/RConn3
  890 D-I/LConn1 -- 890/RConn1
  890 D-I/LConn2 -- 890/RConn2
  890 D-I/LConn3 -- 890/RConn3
  858-834/LConn2 -- 858 D-PQ/LConn2 -- 858/RConn2
  Load Flow Bus22/LConn3 -- 858 D-Z/LConn3 -- 832-858/RConn3
  Load Flow Bus22/LConn1 -- 858 D-Z/LConn1 -- 832-858/RConn1
  858/LConn3 -- Load Flow Bus22/RConn3
  Load Flow Bus22/LConn2 -- 858 D-Z/LConn2 -- 832-858/RConn2
  858/LConn1 -- Load Flow Bus22/RConn1
  858-834/LConn1 -- 858 D-PQ/LConn1 -- 858-864/LConn1 -- 858 Y-PQ/LConn1 -- 858/RConn1
  858/LConn2 -- Load Flow Bus22/RConn2
  858-834/LConn3 -- 858 D-PQ/LConn3 -- 858/RConn3
  Load Flow Bus25/LConn3 -- 860 D-Z/LConn3 -- 834-860/RConn3
  834-860/LConn1 -- 834 D-Z/LConn1 -- 834-842/LConn1 -- 834/RConn1
  834/LConn2 -- Load Flow Bus24/RConn2
  860/LConn3 -- Load Flow Bus25/RConn3
  834/LConn3 -- Load Flow Bus24/RConn3
  860/LConn1 -- Load Flow Bus25/RConn1
  Load Flow Bus24/LConn2 -- 834 D-PQ/LConn2 -- 858-834/RConn2
  Load Flow Bus24/LConn1 -- 834 D-PQ/LConn1 -- 858-834/RConn1
  Load Flow Bus24/LConn3 -- 834 D-PQ/LConn3 -- 858-834/RConn3
  834/LConn1 -- Load Flow Bus24/RConn1
  Load Flow Bus25/LConn2 -- 860 D-Z/LConn2 -- 834-860/RConn2
  860/LConn2 -- Load Flow Bus25/RConn2
  834-860/LConn3 -- 834 D-Z/LConn3 -- 834-842/LConn3 -- 834/RConn3
  834-860/LConn2 -- 834 D-Z/LConn2 -- 834-842/LConn2 -- 834/RConn2
  Load Flow Bus25/LConn1 -- 860 D-Z/LConn1 -- 834-860/RConn1
  832 D-Z/LConn1 -- 832/RConn1 -- XF-10 24.9kV / 4.16kV/LConn1 -- 832-858/LConn1
  832 D-Z/LConn2 -- 832/RConn2 -- XF-10 24.9kV / 4.16kV/LConn2 -- 832-858/LConn2
  Load Flow Bus26/LConn1 -- 836 D-PQ/LConn1 -- 860-836/RConn1
  Load Flow Bus26/LConn2 -- 836 D-PQ/LConn2 -- 860-836/RConn2
  836/LConn3 -- Load Flow Bus26/RConn3
  836/LConn1 -- Load Flow Bus26/RConn1
  Load Flow Bus26/LConn3 -- 836 D-PQ/LConn3 -- 860-836/RConn3
  836/LConn2 -- Load Flow Bus26/RConn2
  860-836/LConn1 -- 860 D-PQ/LConn1 -- 860 Y-PQ/LConn1 -- 860/RConn1
  860-836/LConn2 -- 860 D-PQ/LConn2 -- 860 Y-PQ/LConn2 -- 860/RConn2
  860-836/LConn3 -- 860 D-PQ/LConn3 -- 860 Y-PQ/LConn3 -- 860/RConn3
  Load Flow Bus27/LConn1 -- 836-840/RConn1 -- 840 D-I/LConn1
  Load Flow Bus27/LConn2 -- 836-840/RConn2 -- 840 D-I/LConn2
  840/LConn1 -- Load Flow Bus27/RConn1
  840/LConn2 -- Load Flow Bus27/RConn2
  Load Flow Bus27/LConn3 -- 836-840/RConn3 -- 840 D-I/LConn3
  840/LConn3 -- Load Flow Bus27/RConn3
  836-840/LConn1 -- 836/RConn1 -- 836-862/LConn1 -- 836 D-I/LConn1
  836-840/LConn2 -- 836-862/LConn2 -- 836/RConn2 -- 836 D-I/LConn2
  836-840/LConn3 -- 836-862/LConn3 -- 836/RConn3 -- 836 D-I/LConn3
  840 Y-I/LConn1 -- 840/RConn1
  840 Y-I/LConn2 -- 840/RConn2
  840 Y-I/LConn3 -- 840/RConn3
  Load Flow Bus30/LConn1 -- 834-842/RConn1
  842/LConn2 -- Load Flow Bus30/RConn2
  842/LConn3 -- Load Flow Bus30/RConn3
  Load Flow Bus30/LConn2 -- 834-842/RConn2
  Load Flow Bus30/LConn3 -- 834-842/RConn3
  842/LConn1 -- Load Flow Bus30/RConn1
  Load Flow Bus31/LConn2 -- 844 Y-PQ/LConn2 -- 842-844/RConn2
  844/LConn2 -- Load Flow Bus31/RConn2
  Load Flow Bus31/LConn1 -- 844 Y-PQ/LConn1 -- 842-844/RConn1
  844/LConn1 -- Load Flow Bus31/RConn1
  842-844/LConn1 -- 842 Y-PQ/LConn1 -- 842/RConn1
  842-844/LConn2 -- 842 Y-PQ/LConn2 -- 842/RConn2
  842-844/LConn3 -- 842 Y-PQ/LConn3 -- 842/RConn3
  Load Flow Bus32/LConn2 -- 844-846/RConn2 -- 846 Y-PQ/LConn2
  846/LConn2 -- Load Flow Bus32/RConn2
  Load Flow Bus32/LConn1 -- 844-846/RConn1 -- 846 Y-PQ/LConn1
  846/LConn1 -- Load Flow Bus32/RConn1
  844-846/LConn1 -- 844 Y-PQ1/LConn1 -- 844 Y-Z1/LConn1 -- 844 Y-Z/LConn1 -- 844/RConn1
  844-846/LConn2 -- 844 Y-PQ1/LConn2 -- 844 Y-Z1/LConn2 -- 844 Y-Z/LConn2 -- 844/RConn2
  844-846/LConn3 -- 844 Y-PQ1/LConn3 -- 844 Y-Z1/LConn3 -- 844 Y-Z/LConn3 -- 844/RConn3
  Load Flow Bus33/LConn2 -- 848 Y-PQ/LConn2 -- 846-848/RConn2
  848/LConn2 -- Load Flow Bus33/RConn2
  Load Flow Bus33/LConn1 -- 848 Y-PQ/LConn1 -- 846-848/RConn1
  848/LConn1 -- Load Flow Bus33/RConn1
  846-848/LConn1 -- 846 Y-PQ1/LConn1 -- 846/RConn1
  846-848/LConn2 -- 846 Y-PQ1/LConn2 -- 846/RConn2
  846-848/LConn3 -- 846 Y-PQ1/LConn3 -- 846/RConn3
  848 D-PQ/LConn1 -- 848 D-Z/LConn1 -- 848/RConn1
  848 D-PQ/LConn2 -- 848 D-Z/LConn2 -- 848/RConn2
  848 D-PQ/LConn3 -- 848 D-Z/LConn3 -- 848/RConn3
  Load Flow Bus20/LConn1 -- XF-10 24.9kV / 4.16kV/RConn1
  Load Flow Bus20/LConn2 -- XF-10 24.9kV / 4.16kV/RConn2
  Load Flow Bus20/LConn3 -- XF-10 24.9kV / 4.16kV/RConn3
  826 Y-I/LConn1 -- Load Flow Bus10/LConn1 -- 824-826/RConn1
  856 Y-PQ/LConn1 -- Load Flow Bus17/LConn1 -- 854-856/RConn1
  838 Y-PQ/LConn1 -- 862-838/RConn1 -- Load Flow Bus29/LConn1
  Ground1/LConn1 -- 810 Y-I/RConn1
  Ground2/LConn1 -- 818 Y-Z/RConn1
  Ground3/LConn1 -- 820 Y-Z/RConn1
  Ground4/LConn1 -- 820 Y-PQ/RConn1
  Ground5/LConn1 -- 822 Y-PQ/RConn1
  862-838/LConn1 -- 862 Y-PQ/LConn1 -- Load Flow Bus36/RConn1
  Ground8/LConn1 -- 824 Y-I/RConn1
  Ground9/LConn1 -- 826 Y-I/RConn1
  842-844/RConn3 -- 844 Y-PQ/LConn3 -- Load Flow Bus31/LConn3
  Load Flow Bus31/RConn3 -- 844/LConn3
  844-846/RConn3 -- 846 Y-PQ/LConn3 -- Load Flow Bus32/LConn3
  Load Flow Bus32/RConn3 -- 846/LConn3
  846-848/RConn3 -- 848 Y-PQ/LConn3 -- Load Flow Bus33/LConn3
  Load Flow Bus33/RConn3 -- 848/LConn3
  Ground10/LConn1 -- 854 Y-PQ/RConn1
  Ground11/LConn1 -- 856 Y-PQ/RConn1
  Ground12/LConn1 -- 858 Y-PQ/RConn1
  Ground13/LConn1 -- 864 Y-PQ/RConn1
  864 Y-PQ/LConn1 -- 858-864/RConn1 -- Load Flow Bus23/LConn1
  Ground14/LConn1 -- 862 Y-PQ/RConn1
  Ground15/LConn1 -- 838 Y-PQ/RConn1
  Load Flow Bus/RConn1 -- 800-802/LConn1
  Load Flow Bus/RConn2 -- 800-802/LConn2
  Load Flow Bus/RConn3 -- 800-802/LConn3
  Load Flow Bus2/RConn1 -- 806-808/LConn1
  Load Flow Bus2/RConn2 -- 806-808/LConn2
  Load Flow Bus2/RConn3 -- 806-808/LConn3
  812-814/LConn1 -- Load Flow Bus4/RConn1
  812-814/LConn2 -- Load Flow Bus4/RConn2
  812-814/LConn3 -- Load Flow Bus4/RConn3
  814-850/LConn1 -- Load Flow Bus5/RConn1
  814-850/LConn2 -- Load Flow Bus5/RConn2
  814-850/LConn3 -- Load Flow Bus5/RConn3
  850-816/LConn1 -- Load Flow Bus7/RConn1
  850-816/LConn2 -- Load Flow Bus7/RConn2
  850-816/LConn3 -- Load Flow Bus7/RConn3
  830/LConn1 -- Load Flow Bus15/RConn1
  830/LConn2 -- Load Flow Bus15/RConn2
  830/LConn3 -- Load Flow Bus15/RConn3
  830-854/LConn1 -- 830 D-Z/LConn1 -- 830/RConn1
  830-854/LConn2 -- 830 D-Z/LConn2 -- 830/RConn2
  830-854/LConn3 -- 830 D-Z/LConn3 -- 830/RConn3
  852-832/LConn1 -- Load Flow Bus18/RConn1
  852-832/LConn2 -- Load Flow Bus18/RConn2
  852-832/LConn3 -- Load Flow Bus18/RConn3
  888-890/LConn1 -- Load Flow Bus20/RConn1
  888-890/LConn2 -- Load Flow Bus20/RConn2
  888-890/LConn3 -- Load Flow Bus20/RConn3
  808-810/RConn1 -- 810 Y-I/LConn1 -- Load Flow Bus6/LConn1
  816-818/RConn1 -- Load Flow Bus11/LConn1
  832 D-Z/LConn3 -- 832/RConn3 -- XF-10 24.9kV / 4.16kV/LConn3 -- 832-858/LConn3
  Ground/LConn1 -- 808 Y-I/RConn1
  Load Flow Bus36/LConn1 -- 836-862/RConn2
  Load Flow Bus34/LConn1 -- 836-862/RConn1
  Load Flow Bus35/LConn1 -- 836-862/RConn3
